simulink library "xbsIndex_r4"  (Simulink 7.1)
(part 6 of 9)

      settings: CopyFcn=xlBlockMoveCallback(gcbh);  DeleteFcn=xlDestroyGui(gcbh);  ModelCloseFcn=xlDestroyGui(gcbh);  PreSaveFcn=xlBlockPreSaveCallback(gcbh);  PostSaveFcn=xlBlockPostSaveCallback(gcbh);  DestroyFcn=xlDestroyGui(gcbh);  OpenFcn=xlOpenGui(gcbh, 'lfsr_gui.xml', @lfsrenablement, -1)  CloseFcn=xlDestroyGui(gcbh);  MoveFcn=xlBlockMoveCallback(gcbh);
      mask Help: eval('');xlDoc('-book','sysgen','-topic','LFSR');
      mask StyleString: edit,popup(Fibonacci|Galois),edit,popup(XOR|XNOR),edit,edit,edit,edit,checkbox,edit,checkbox,edit,checkbox,edit,checkbox,edit,checkbox,edit,popup(Signed  (2's comp)|Unsigned),edit,edit,checkbox,edit,checkbox,edit,edit,checkbox,edit,edit,edit,edit,edit,edit,edit,edit,edit
      mask Display:
      | fprintf('','COMMENT: begin icon graphics');
      | patch([0 60 60 0 0 ],[0 0 60 60 0 ],[0.77 0.82 0.91 ]);
      | plot([0 60 60 0 0 ],[0 0 60 60 0 ]);
      | patch([12.2 23.76 31.76 39.76 47.76 31.76 20.2 12.2 ],[38.88 38.88 46.88 38.88 46.88 46.88 46.88 38.88 ],[1 1 1 ]);
      | patch([20.2 31.76 23.76 12.2 20.2 ],[30.88 30.88 38.88 38.88 30.88 ],[0.931 0.946 0.973 ]);
      | patch([12.2 23.76 31.76 20.2 12.2 ],[22.88 22.88 30.88 30.88 22.88 ],[1 1 1 ]);
      | patch([20.2 47.76 39.76 31.76 23.76 12.2 20.2 ],[14.88 14.88 22.88 14.88 22.88 22.88 14.88 ],[0.931 0.946 0.973 ]);
      | fprintf('','COMMENT: end icon graphics');
      | fprintf('','COMMENT: begin icon text');
      | color('black');port_label('output',1,'dout');
      | fprintf('','COMMENT: end icon text');
  Logical : S-Function  LoadFcn=xlBlockLoadCallback(gcbh);  FunctionName=sysgen  Parameters=ptable_  EnableBusSupport=off  mask(Xilinx Logical Block Block){logical_function_sgadvanced=, logical_function=AND, inputs=2, en_sgadvanced=, en=off, latency=0, precision_sgadvanced=, precision=Full, arith_type_sgadvanced=, arith_type=Unsigned, n_bits=16, bin_pt=0, align_bp_sgadvanced=, align_bp=on, dbl_ovrd_sgadvanced=, dbl_ovrd=off, xl_use_area_sgadvanced=, xl_use_area=off, xl_area=[0,0,0,0,0,0,0], overflow=, quantization=, has_advanced_control=0, sggui_pos=-1,-1,-1,-1, block_type=logical, block_version=, sg_icon_stat=55,60,2,1,white,blue,0,83a4b621,right,,[ ],[ ], sg_mask_display=|, sg_list_contents=, sg_blockgui_xml=}
      mask sg_mask_display=|
      | fprintf('','COMMENT: begin icon graphics');
      | patch([0 55 55 0 0 ],[0 0 60 60 0 ],[0.77 0.82 0.91 ]);
      | plot([0 55 55 0 0 ],[0 0 60 60 0 ]);
      | patch([11.425 21.54 28.54 35.54 42.54 28.54 18.425 11.425 ],[37.77 37.77 44.77 37.77 44.77 44.77 44.77 37.77 ],[1 1 1 ]);
      | patch([18.425 28.54 21.54 11.425 18.425 ],[30.77 30.77 37.77 37.77 30.77 ],[0.931 0.946 0.973 ]);
      | patch([11.425 21.54 28.54 18.425 11.425 ],[23.77 23.77 30.77 30.77 23.77 ],[1 1 1 ]);
      | patch([18.425 42.54 35.54 28.54 21.54 11.425 18.425 ],[16.77 16.77 23.77 16.77 23.77 23.77 16.77 ],[0.931 0.946 0.973 ]);
      | fprintf('','COMMENT: end icon graphics');
      | fprintf('','COMMENT: begin icon text');
      |
      |
      |
      | color('black');disp('and');
      | fprintf('','COMMENT: end icon text');
      mask prompts: logical_function_sgadvanced ""; logical_function "Logical function"; inputs "Number of inputs"; en_sgadvanced ""; en "Provide enable port"; precision_sgadvanced ""; arith_type_sgadvanced ""; arith_type "Output Type"; n_bits "Number of bits"; bin_pt "Binary point"; align_bp_sgadvanced ""; align_bp "Align binary point"; dbl_ovrd_sgadvanced ""; dbl_ovrd "Override with doubles"; xl_use_area_sgadvanced ""; xl_use_area "Define FPGA area for resource estimation"; xl_area "FPGA area [slices, FFs, BRAMs, LUTs, IOBs, emb. mults, TBUFs]"; overflow ""; quantization ""; has_advanced_control ""; sggui_pos ""; block_type ""; block_version ""; sg_icon_stat ""; sg_mask_display ""; sg_list_contents ""; sg_blockgui_xml ""
      mask help: Xilinx Logical Block
      mask init:
      | try
      |   tmp_gcb = gcb;
      |   tmp_gcbh = gcbh;
      |   if (strcmp('SysGenIndex',get_param(bdroot(tmp_gcbh),'tag')) && ~isempty(regexp(bdroot(tmp_gcb), '^xbs', 'once')))
      |     return;
      |   end;
      |   xlMungeMaskParams;
      |   block_config = 'sysgen_blockset:Logical_config';
      | 
      |   block_type='logical';
      | 
      |   serialized_declarations = '{''arith_type''=>''Int'',''bin_pt''=>''Int'',''en''=>''Int'',''inputs''=>''Int'',''latency''=>''Int'',''logical_function''=>''Int'',''n_bits''=>''Int'',''precision''=>''Int'',''sim_engine''=>''Int'',''sysgen_root''=>''String'',''block_type''=>''String''}';
      |   xllogical_init();
      |   ptable_ = xlblockprep(get_param(tmp_gcb, 'MaskWSVariables'));
      |   try
      |     xlBlockMoveCallback(tmp_gcbh);
      |   catch 
      |      clear global xl_updateicon_recursion_guard;
      |   end;
      | catch
      |   global dbgsysgen;
      |   if(~isempty(dbgsysgen) && dbgsysgen)
      |     e = regexprep(lasterr, '\n', '\nError: ');
      |     disp(['Error: While running MaskInit code on block ' tmp_gcb ': ' e]);
      |     error(e);
      |   end
      | end
      settings: CopyFcn=xlBlockMoveCallback(gcbh);  DeleteFcn=xlDestroyGui(gcbh);  ModelCloseFcn=xlDestroyGui(gcbh);  PreSaveFcn=xlBlockPreSaveCallback(gcbh);  PostSaveFcn=xlBlockPostSaveCallback(gcbh);  DestroyFcn=xlDestroyGui(gcbh);  OpenFcn=xlOpenGui(gcbh, 'logical_gui.xml', @logicalenablement, -1)  CloseFcn=xlDestroyGui(gcbh);  MoveFcn=xlBlockMoveCallback(gcbh);
      mask Help: eval('');xlDoc('-book','sysgen','-topic','Logical');
      mask StyleString: edit,popup(AND|NAND|OR|NOR|XOR|XNOR),edit,edit,checkbox,edit,edit,popup(Full|User Defined),edit,popup(Signed  (2's comp)|Unsigned),edit,edit,edit,checkbox,edit,checkbox,edit,checkbox,edit,edit,edit,edit,edit,edit,edit,edit,edit,edit,edit
      mask Display:
      | fprintf('','COMMENT: begin icon graphics');
      | patch([0 55 55 0 0 ],[0 0 60 60 0 ],[0.77 0.82 0.91 ]);
      | plot([0 55 55 0 0 ],[0 0 60 60 0 ]);
      | patch([11.425 21.54 28.54 35.54 42.54 28.54 18.425 11.425 ],[37.77 37.77 44.77 37.77 44.77 44.77 44.77 37.77 ],[1 1 1 ]);
      | patch([18.425 28.54 21.54 11.425 18.425 ],[30.77 30.77 37.77 37.77 30.77 ],[0.931 0.946 0.973 ]);
      | patch([11.425 21.54 28.54 18.425 11.425 ],[23.77 23.77 30.77 30.77 23.77 ],[1 1 1 ]);
      | patch([18.425 42.54 35.54 28.54 21.54 11.425 18.425 ],[16.77 16.77 23.77 16.77 23.77 23.77 16.77 ],[0.931 0.946 0.973 ]);
      | fprintf('','COMMENT: end icon graphics');
      | fprintf('','COMMENT: begin icon text');
      | 
      | 
      | 
      | color('black');disp('and');
      | fprintf('','COMMENT: end icon text');
  MCode : S-Function  LoadFcn=xlBlockLoadCallback(gcbh);  FunctionName=sysgen  Parameters=ptable_  EnableBusSupport=off  mask(Xilinx MCode Block Block){infoedit=Pass input values to a MATLAB function for evaluation in Xilinx fixed-point type. The input ports of the block are input arguments of the function. The output ports of the block are output arguments of the function., mfname=xlmax, explicit_period_sgadvanced=, explicit_period=off, period=1, inputsTable=, outputsTable=, dbl_ovrd_sgadvanced=, dbl_ovrd=off, enable_stdout_sgadvanced=, enable_stdout=off, enable_debug_sgadvanced=, enable_debug=off, xl_use_area_sgadvanced=, xl_use_area=off, xl_area=[0,0,0,0,0,0,0], mfilecontent=, suppress_output=on, defparams={}, hide_port_list={}, has_advanced_control=0, sggui_pos=-1,-1,-1,-1, block_type=mcode, block_version=, sg_icon_stat=65,62,2,1,white,blue,0,0442c75a,right,,[ ],[ ], sg_mask_display=|, sg_list_contents=, sg_blockgui_xml=}
      mask sg_mask_display=|
      | fprintf('','COMMENT: begin icon graphics');
      | patch([0 65 65 0 0 ],[0 0 62 62 0 ],[0.77 0.82 0.91 ]);
      | plot([0 65 65 0 0 ],[0 0 62 62 0 ]);
      | patch([14.2 25.76 33.76 41.76 49.76 33.76 22.2 14.2 ],[39.88 39.88 47.88 39.88 47.88 47.88 47.88 39.88 ],[1 1 1 ]);
      | patch([22.2 33.76 25.76 14.2 22.2 ],[31.88 31.88 39.88 39.88 31.88 ],[0.931 0.946 0.973 ]);
      | patch([14.2 25.76 33.76 22.2 14.2 ],[23.88 23.88 31.88 31.88 23.88 ],[1 1 1 ]);
      | patch([22.2 49.76 41.76 33.76 25.76 14.2 22.2 ],[15.88 15.88 23.88 15.88 23.88 23.88 15.88 ],[0.931 0.946 0.973 ]);
      | fprintf('','COMMENT: end icon graphics');
      | fprintf('','COMMENT: begin icon text');
      | color('black');port_label('input',1,'x');
      | color('black');port_label('input',2,'y');
      | color('black');port_label('output',1,'z');
      | color('black');disp('\bf{xlmax}','texmode','on');
      | fprintf('','COMMENT: end icon text');
      mask prompts: infoedit ""; mfname "MATLAB function"; explicit_period_sgadvanced ""; explicit_period "Specify explicit sample period"; period ""; inputsTable ""; outputsTable ""; dbl_ovrd_sgadvanced ""; dbl_ovrd "Override with doubles"; enable_stdout_sgadvanced ""; enable_stdout "Enable printing with disp"; enable_debug_sgadvanced ""; enable_debug "Enable MATLAB debugging (slows simulation)"; xl_use_area_sgadvanced ""; xl_use_area "Define FPGA area for resource estimation"; xl_area "FPGA area [slices, FFs, BRAMs, LUTs, IOBs, emb. mults, TBUFs]"; mfilecontent ""; suppress_output ""; defparams ""; hide_port_list ""; has_advanced_control ""; sggui_pos ""; block_type ""; block_version ""; sg_icon_stat ""; sg_mask_display ""; sg_list_contents ""; sg_blockgui_xml ""
      mask help: Pass input values to a MATLAB function for evaluation in Xilinx fixed-point type. The input ports of the block are input arguments of the function. The output ports of the block are output arguments of the function.
      mask init:
      | try
      |   tmp_gcb = gcb;
      |   tmp_gcbh = gcbh;
      |   if (strcmp('SysGenIndex',get_param(bdroot(tmp_gcbh),'tag')) && ~isempty(regexp(bdroot(tmp_gcb), '^xbs', 'once')))
      |     return;
      |   end;
      |   xlMungeMaskParams;
      |   block_config = 'sysgen_blockset:mcode_block_config';
      | 
      |   block_type='mcode';
      | 
      |   serialized_declarations = '{''block_fullname''=>''String'',''bool_vec_lens''=>''IntVector'',''bool_vec_names''=>''StringVector'',''bool_vec_values''=>''IntVector'',''dbl_vec_lens''=>''IntVector'',''dbl_vec_names''=>''StringVector'',''dbl_vec_values''=>''DoubleVector'',''defparams''=>''Struct'',''drawport''=>''String'',''enable_debug''=>''Int'',''enable_stdout''=>''Int'',''error_msgs''=>''StringVector'',''explicitClk''=>''Int'',''explicit_period''=>''Int'',''hide_port_list''=>''StringVector'',''icontext''=>''String'',''mfile_dir''=>''String'',''mfilecontent''=>''String'',''mfilename''=>''String'',''mfname''=>''String'',''param_names_bool''=>''StringVector'',''param_names_double''=>''StringVector'',''param_values_bool''=>''IntVector'',''param_values_double''=>''DoubleVector'',''period''=>''Double'',''sgpfilename''=>''String'',''sysgen_root''=>''String'',''block_type''=>''String''}';
      |   xlmcode_init();
      |   ptable_ = xlblockprep(get_param(tmp_gcb, 'MaskWSVariables'));
      |   try
      |     xlBlockMoveCallback(tmp_gcbh);
      |   catch 
      |      clear global xl_updateicon_recursion_guard;
      |   end;
      | catch
      |   global dbgsysgen;
      |   if(~isempty(dbgsysgen) && dbgsysgen)
      |     e = regexprep(lasterr, '\n', '\nError: ');
      |     disp(['Error: While running MaskInit code on block ' tmp_gcb ': ' e]);
      |     error(e);
      |   end
      | end
      settings: CopyFcn=xlBlockMoveCallback(gcbh);  DeleteFcn=xlDestroyGui(gcbh);  ModelCloseFcn=xlDestroyGui(gcbh);  PreSaveFcn=xlBlockPreSaveCallback(gcbh);  PostSaveFcn=xlBlockPostSaveCallback(gcbh);  DestroyFcn=xlDestroyGui(gcbh);  OpenFcn=xlOpenGui(gcbh, 'mcode_gui.xml', @mcodeenablement, @mcodeaction)  CloseFcn=xlDestroyGui(gcbh);  MoveFcn=xlBlockMoveCallback(gcbh);
      mask Help: eval('');xlDoc('-book','sysgen','-topic','MCode');
      mask Display:
      | fprintf('','COMMENT: begin icon graphics');
      | patch([0 65 65 0 0 ],[0 0 62 62 0 ],[0.77 0.82 0.91 ]);
      | plot([0 65 65 0 0 ],[0 0 62 62 0 ]);
      | patch([14.2 25.76 33.76 41.76 49.76 33.76 22.2 14.2 ],[39.88 39.88 47.88 39.88 47.88 47.88 47.88 39.88 ],[1 1 1 ]);
      | patch([22.2 33.76 25.76 14.2 22.2 ],[31.88 31.88 39.88 39.88 31.88 ],[0.931 0.946 0.973 ]);
      | patch([14.2 25.76 33.76 22.2 14.2 ],[23.88 23.88 31.88 31.88 23.88 ],[1 1 1 ]);
      | patch([22.2 49.76 41.76 33.76 25.76 14.2 22.2 ],[15.88 15.88 23.88 15.88 23.88 23.88 15.88 ],[0.931 0.946 0.973 ]);
      | fprintf('','COMMENT: end icon graphics');
      | fprintf('','COMMENT: begin icon text');
      | color('black');port_label('input',1,'x');
      | color('black');port_label('input',2,'y');
      | color('black');port_label('output',1,'z');
      | color('black');disp('\bf{xlmax}','texmode','on');
      | fprintf('','COMMENT: end icon text');
  ModelSim : S-Function  LoadFcn=xlBlockLoadCallback(gcbh);  FunctionName=sysgen  Parameters=ptable_  EnableBusSupport=off  mask(ModelSim HDL Co-Simulation Interface Block){infoedit=Allow other blocks to schedule HDL co-simulation tasks.<br><br>Note that selecting "Skip compilation" when inappropriate can cause simulation errors and failures. Please refer to the block help for details., dir=./modelsim, waveform_sgadvanced=, waveform=on, leave_open_sgadvanced=, leave_open=on, skip_compile_sgadvanced=, skip_compile=off, use_unisim_sgadvanced=, use_unisim=off, use_ver_xilinxcorelib_sgadvanced=, use_ver_xilinxcorelib=off, custom_scripts_sgadvanced=, custom_scripts=off, pre_comp_script=, vsim_script=, post_vsim_script=, startup_timeout=40, has_advanced_control=0, sggui_pos=-1,-1,-1,-1, block_type=hdlcosim, block_version=, sg_icon_stat=65,56,0,0,blue,white,0,efd5b770,right,,[ ],[ ], sg_mask_display=|, sg_list_contents=, sg_blockgui_xml=}
      mask sg_mask_display=|
      | fprintf('','COMMENT: begin icon graphics');
      | patch([0 65 65 0 0 ],[0 0 56 56 0 ],[1 1 1 ]);
      | plot([0 65 65 0 0 ],[0 0 56 56 0 ]);
      | patch([14.2 25.76 33.76 41.76 49.76 33.76 22.2 14.2 ],[36.88 36.88 44.88 36.88 44.88 44.88 44.88 36.88 ],[0.839 0.874 0.937 ]);
      | patch([22.2 33.76 25.76 14.2 22.2 ],[28.88 28.88 36.88 36.88 28.88 ],[0.77 0.82 0.91 ]);
      | patch([14.2 25.76 33.76 22.2 14.2 ],[20.88 20.88 28.88 28.88 20.88 ],[0.839 0.874 0.937 ]);
      | patch([22.2 49.76 41.76 33.76 25.76 14.2 22.2 ],[12.88 12.88 20.88 12.88 20.88 20.88 12.88 ],[0.77 0.82 0.91 ]);
      | fprintf('','COMMENT: end icon graphics');
      | fprintf('','COMMENT: begin icon text');
      |
      | fprintf('','COMMENT: end icon text');fprintf('ModelSim');
      mask prompts: infoedit ""; dir "Run co-simulation in directory:"; waveform_sgadvanced ""; waveform "Open waveform viewer"; leave_open_sgadvanced ""; leave_open "Leave ModelSim open at end of simulation"; skip_compile_sgadvanced ""; skip_compile "Skip compilation (use previous results)"; use_unisim_sgadvanced ""; use_unisim "Include Verilog unisim library"; use_ver_xilinxcorelib_sgadvanced ""; use_ver_xilinxcorelib "Include Verilog XILINXCORELIB library"; custom_scripts_sgadvanced ""; custom_scripts "Add custom scripts"; pre_comp_script "Script to run before starting compilation:"; vsim_script "Script to run in place of  "vsim":"; post_vsim_script "Script to run after "vsim":"; startup_timeout ""; has_advanced_control ""; sggui_pos ""; block_type ""; block_version ""; sg_icon_stat ""; sg_mask_display ""; sg_list_contents ""; sg_blockgui_xml ""
      mask help:
      | Allow other blocks to schedule HDL co-simulation tasks.
      |
      | Note that selecting "Skip compilation" when inappropriate can cause simulation errors and failures. Please refer to the block help for details.
      mask init:
      | try
      |   tmp_gcb = gcb;
      |   tmp_gcbh = gcbh;
      |   if (strcmp('SysGenIndex',get_param(bdroot(tmp_gcbh),'tag')) && ~isempty(regexp(bdroot(tmp_gcb), '^xbs', 'once')))
      |     return;
      |   end;
      |   xlMungeMaskParams;
      |   block_config = 'Sysgen:hdlcosim_block_config';
      | 
      |   block_type='hdlcosim';
      | 
      |   serialized_declarations = '{''binDir''=>''String'',''custom_scripts''=>''Int'',''dir''=>''String'',''engineDll''=>''String'',''leave_open''=>''Int'',''mdlPath''=>''String'',''period''=>''Double'',''post_vsim_script''=>''String'',''pre_comp_script''=>''String'',''screenSize''=>''DoubleVector'',''sim_status''=>''String'',''skip_compile''=>''Int'',''startup_timeout''=>''Int'',''use_unisim''=>''Int'',''use_ver_xilinxcorelib''=>''Int'',''vsim_script''=>''String'',''waveform''=>''Int'',''block_type''=>''String''}';
      |   xlhdlcosim_init();
      |   ptable_ = xlblockprep(get_param(tmp_gcb, 'MaskWSVariables'));
      |   try
      |     xlBlockMoveCallback(tmp_gcbh);
      |   catch 
      |      clear global xl_updateicon_recursion_guard;
      |   end;
      | catch
      |   global dbgsysgen;
      |   if(~isempty(dbgsysgen) && dbgsysgen)
      |     e = regexprep(lasterr, '\n', '\nError: ');
      |     disp(['Error: While running MaskInit code on block ' tmp_gcb ': ' e]);
      |     error(e);
      |   end
      | end
      settings: CopyFcn=xlBlockMoveCallback(gcbh);  DeleteFcn=xlDestroyGui(gcbh);  ModelCloseFcn=xlDestroyGui(gcbh);  PreSaveFcn=xlBlockPreSaveCallback(gcbh);  PostSaveFcn=xlBlockPostSaveCallback(gcbh);  DestroyFcn=xlDestroyGui(gcbh);  OpenFcn=xlOpenGui(gcbh, 'hdlcosim_gui.xml', @hdlcosimenablement, -1)  CloseFcn=xlDestroyGui(gcbh);  MoveFcn=xlBlockMoveCallback(gcbh);
      mask Help: eval('');xlDoc('-book','sysgen','-topic','ModelSim');
      mask Display:
      | fprintf('','COMMENT: begin icon graphics');
      | patch([0 65 65 0 0 ],[0 0 56 56 0 ],[1 1 1 ]);
      | plot([0 65 65 0 0 ],[0 0 56 56 0 ]);
      | patch([14.2 25.76 33.76 41.76 49.76 33.76 22.2 14.2 ],[36.88 36.88 44.88 36.88 44.88 44.88 44.88 36.88 ],[0.839 0.874 0.937 ]);
      | patch([22.2 33.76 25.76 14.2 22.2 ],[28.88 28.88 36.88 36.88 28.88 ],[0.77 0.82 0.91 ]);
      | patch([14.2 25.76 33.76 22.2 14.2 ],[20.88 20.88 28.88 28.88 20.88 ],[0.839 0.874 0.937 ]);
      | patch([22.2 49.76 41.76 33.76 25.76 14.2 22.2 ],[12.88 12.88 20.88 12.88 20.88 20.88 12.88 ],[0.77 0.82 0.91 ]);
      | fprintf('','COMMENT: end icon graphics');
      | fprintf('','COMMENT: begin icon text');
      | 
      | fprintf('','COMMENT: end icon text');fprintf('ModelSim');
  Mult : S-Function  LoadFcn=xlBlockLoadCallback(gcbh);  FunctionName=sysgen  Parameters=ptable_  EnableBusSupport=off  mask(Xilinx Multiplier Block){infoedit=Hardware notes: To check for the optimum internal pipeline stages of the dedicated multiplier you must select 'Test for optimum pipelining'.<br><br>Optimization Goal: For implementation into device fabric (LUTs), the Speed or Area optimization will take effect only if it's supported by IP for the particular device family. Otherwise, the results will be identical regardless of the selection., precision_sgadvanced=, precision=Full, arith_type_sgadvanced=, arith_type=Signed  (2's comp), n_bits=16, bin_pt=14, quantization_sgadvanced=, quantization=Truncate, overflow_sgadvanced=, overflow=Wrap, en_sgadvanced=, en=off, latency=3, dbl_ovrd_sgadvanced=, dbl_ovrd=off, use_behavioral_HDL_sgadvanced=, use_behavioral_HDL=off, opt_sgadvanced=, opt=Speed, use_embedded_sgadvanced=, use_embedded=on, optimum_pipeline_sgadvanced=, optimum_pipeline=off, xl_use_area_sgadvanced=, xl_use_area=off, xl_area=[0,0,0,0,0,0,0], pipeline=on, use_rpm=on, placement_style=Triangular, has_advanced_control=0, sggui_pos=-1,-1,-1,-1, block_type=mult, block_version=, sg_icon_stat=55,55,2,1,white,blue,0,7028354c,right,,[ ],[ ], sg_mask_display=|, sg_list_contents=, sg_blockgui_xml=}
      mask sg_mask_display=|
      | fprintf('','COMMENT: begin icon graphics');
      | patch([0 55 55 0 0 ],[0 0 55 55 0 ],[0.77 0.82 0.91 ]);
      | plot([0 55 55 0 0 ],[0 0 55 55 0 ]);
      | patch([11.425 21.54 28.54 35.54 42.54 28.54 18.425 11.425 ],[34.77 34.77 41.77 34.77 41.77 41.77 41.77 34.77 ],[1 1 1 ]);
      | patch([18.425 28.54 21.54 11.425 18.425 ],[27.77 27.77 34.77 34.77 27.77 ],[0.931 0.946 0.973 ]);
      | patch([11.425 21.54 28.54 18.425 11.425 ],[20.77 20.77 27.77 27.77 20.77 ],[1 1 1 ]);
      | patch([18.425 42.54 35.54 28.54 21.54 11.425 18.425 ],[13.77 13.77 20.77 13.77 20.77 20.77 13.77 ],[0.931 0.946 0.973 ]);
      | fprintf('','COMMENT: end icon graphics');
      | fprintf('','COMMENT: begin icon text');
      | color('black');port_label('input',1,'a');
      | color('black');port_label('input',2,'b');
      | color('black');port_label('output',1,'\bfa \times b','texmode','on');
      | color('black');disp('z^{-3}\newline ','texmode','on');
      | color('black');disp(' \n ');
      | fprintf('','COMMENT: end icon text');
      mask prompts: infoedit ""; precision_sgadvanced ""; arith_type_sgadvanced ""; arith_type "Arithmetic type"; n_bits "Number of bits"; bin_pt "Binary point"; quantization_sgadvanced ""; overflow_sgadvanced ""; en_sgadvanced ""; en "Provide enable port"; dbl_ovrd_sgadvanced ""; dbl_ovrd "Override with doubles"; use_behavioral_HDL_sgadvanced ""; use_behavioral_HDL "Use behavioral HDL (otherwise use core)"; opt_sgadvanced ""; opt "Optimize for"; use_embedded_sgadvanced ""; use_embedded "Use embedded multipliers"; optimum_pipeline_sgadvanced ""; optimum_pipeline "Test for optimum pipelining"; xl_use_area_sgadvanced ""; xl_use_area "Define FPGA area for resource estimation"; xl_area "FPGA area [slices, FFs, BRAMs, LUTs, IOBs, emb. mults, TBUFs]"; pipeline ""; use_rpm ""; placement_style ""; has_advanced_control ""; sggui_pos ""; block_type ""; block_version ""; sg_icon_stat ""; sg_mask_display ""; sg_list_contents ""; sg_blockgui_xml ""
      mask help:
      | Hardware notes: To check for the optimum internal pipeline stages of the dedicated multiplier you must select 'Test for optimum pipelining'.
      |
      | Optimization Goal: For implementation into device fabric (LUTs), the Speed or Area optimization will take effect only if it's supported by IP for the particular device family. Otherwise, the results will be identical regardless of the selection.
      mask init:
      | try
      |   tmp_gcb = gcb;
      |   tmp_gcbh = gcbh;
      |   if (strcmp('SysGenIndex',get_param(bdroot(tmp_gcbh),'tag')) && ~isempty(regexp(bdroot(tmp_gcb), '^xbs', 'once')))
      |     return;
      |   end;
      |   xlMungeMaskParams;
      |   block_config = 'sysgen_blockset:Mult_config';
      | 
      |   block_type='mult';
      | 
      |   serialized_declarations = '{''arith_type''=>''Int'',''bin_pt''=>''Int'',''en''=>''Int'',''latency''=>''Int'',''n_bits''=>''Int'',''opt''=>''Int'',''optimum_pipeline''=>''Int'',''overflow''=>''Int'',''precision''=>''Int'',''quantization''=>''Int'',''use_behavioral_HDL''=>''Int'',''use_embedded''=>''Int'',''block_type''=>''String''}';
      |   ptable_ = xlblockprep(get_param(tmp_gcb, 'MaskWSVariables'));
      |   try
      |     xlBlockMoveCallback(tmp_gcbh);
      |   catch 
      |      clear global xl_updateicon_recursion_guard;
      |   end;
      | catch
      |   global dbgsysgen;
      |   if(~isempty(dbgsysgen) && dbgsysgen)
      |     e = regexprep(lasterr, '\n', '\nError: ');
      |     disp(['Error: While running MaskInit code on block ' tmp_gcb ': ' e]);
      |     error(e);
      |   end
      | end
      settings: CopyFcn=xlBlockMoveCallback(gcbh);  DeleteFcn=xlDestroyGui(gcbh);  ModelCloseFcn=xlDestroyGui(gcbh);  PreSaveFcn=xlBlockPreSaveCallback(gcbh);  PostSaveFcn=xlBlockPostSaveCallback(gcbh);  DestroyFcn=xlDestroyGui(gcbh);  OpenFcn=xlOpenGui(gcbh, 'mult_gui.xml', @multenablement, -1)  CloseFcn=xlDestroyGui(gcbh);  MoveFcn=xlBlockMoveCallback(gcbh);
      mask Help: eval('');xlDoc('-book','sysgen','-topic','Mult');
      mask StyleString: edit,edit,popup(Full|User Defined),edit,popup(Signed  (2's comp)|Unsigned),edit,edit,edit,popup(Truncate|Round  (unbiased: +/- Inf)),edit,popup(Wrap|Saturate|Flag as error),edit,checkbox,edit,edit,checkbox,edit,checkbox,edit,popup(Speed|Area),edit,checkbox,edit,checkbox,edit,checkbox,edit,edit,edit,edit,edit,edit,edit,edit,edit,edit,edit,edit
      mask Display:
      | fprintf('','COMMENT: begin icon graphics');
      | patch([0 55 55 0 0 ],[0 0 55 55 0 ],[0.77 0.82 0.91 ]);
      | plot([0 55 55 0 0 ],[0 0 55 55 0 ]);
      | patch([11.425 21.54 28.54 35.54 42.54 28.54 18.425 11.425 ],[34.77 34.77 41.77 34.77 41.77 41.77 41.77 34.77 ],[1 1 1 ]);
      | patch([18.425 28.54 21.54 11.425 18.425 ],[27.77 27.77 34.77 34.77 27.77 ],[0.931 0.946 0.973 ]);
      | patch([11.425 21.54 28.54 18.425 11.425 ],[20.77 20.77 27.77 27.77 20.77 ],[1 1 1 ]);
      | patch([18.425 42.54 35.54 28.54 21.54 11.425 18.425 ],[13.77 13.77 20.77 13.77 20.77 20.77 13.77 ],[0.931 0.946 0.973 ]);
      | fprintf('','COMMENT: end icon graphics');
      | fprintf('','COMMENT: begin icon text');
      | color('black');port_label('input',1,'a');
      | color('black');port_label('input',2,'b');
      | color('black');port_label('output',1,'\bfa \times b','texmode','on');
      | color('black');disp('z^{-3}\newline ','texmode','on');
      | color('black');disp(' \n ');
      | fprintf('','COMMENT: end icon text');
  Multiple Subsystem Generator : S-Function  Tag=xlStitcher  FunctionName=xlpermissive  Parameters=''  EnableBusSupport=off  mask(Xilinx Subsystem Generator Block){infoedit=Multiple Subsystem\nGenerator, ShowPortLabels=, has_advanced_control=0, sggui_pos=-1,-1,-1,-1, block_type=multiple_subsystem_generator, block_version=, sg_icon_stat=65,65,-1,-1,blue,white,0,07734,right,,[ ],[ ], sg_mask_display=|, sg_list_contents=, sg_blockgui_xml=}
      mask sg_mask_display=|
      | fprintf('','COMMENT: begin icon graphics');
      | patch([0 65 65 0 0 ],[0 0 65 65 0 ],[1 1 1 ]);
      | plot([0 65 65 0 0 ],[0 0 65 65 0 ]);
      | patch([11.975 24.98 33.98 42.98 51.98 33.98 20.975 11.975 ],[41.99 41.99 50.99 41.99 50.99 50.99 50.99 41.99 ],[0.839 0.874 0.937 ]);
      | patch([20.975 33.98 24.98 11.975 20.975 ],[32.99 32.99 41.99 41.99 32.99 ],[0.77 0.82 0.91 ]);
      | patch([11.975 24.98 33.98 20.975 11.975 ],[23.99 23.99 32.99 32.99 23.99 ],[0.839 0.874 0.937 ]);
      | patch([20.975 51.98 42.98 33.98 24.98 11.975 20.975 ],[14.99 14.99 23.99 14.99 23.99 23.99 14.99 ],[0.77 0.82 0.91 ]);
      | fprintf('','COMMENT: end icon graphics');
      | fprintf('','COMMENT: begin icon text');
      | fprintf('','COMMENT: end icon text');
      mask prompts: infoedit ""; ShowPortLabels ""; has_advanced_control ""; sggui_pos ""; block_type ""; block_version ""; sg_icon_stat ""; sg_mask_display ""; sg_list_contents ""; sg_blockgui_xml ""
      mask help: Multiple Subsystem\nGenerator
      mask init:
      | try
      |   tmp_gcb = gcb;
      |   tmp_gcbh = gcbh;
      |   if (strcmp('SysGenIndex',get_param(bdroot(tmp_gcbh),'tag')) && ~isempty(regexp(bdroot(tmp_gcb), '^xbs', 'once')))
      |     return;
      |   end;
      |   xlMungeMaskParams;
      | 
      |   block_type='multiple_subsystem_generator';
      | 
      |   serialized_declarations = '{''block_type''=>''String''}';
      |   ptable_ = xlblockprep(get_param(tmp_gcb, 'MaskWSVariables'));
      |   try
      |     xlBlockMoveCallback(tmp_gcbh);
      |   catch 
      |      clear global xl_updateicon_recursion_guard;
      |   end;
      | catch
      |   global dbgsysgen;
      |   if(~isempty(dbgsysgen) && dbgsysgen)
      |     e = regexprep(lasterr, '\n', '\nError: ');
      |     disp(['Error: While running MaskInit code on block ' tmp_gcb ': ' e]);
      |     error(e);
      |   end
      | end
      settings: CopyFcn=xlBlockMoveCallback(gcbh);  OpenFcn=xldesignStitcher(gcbh);  MoveFcn=xlBlockMoveCallback(gcbh);
      settings: DeleteFcn=|
      | hndls = xlfindsysgenfig(gcb,'stitcher_gui');
      | if (hndls)
      |   close(hndls(1));
      | end
      mask Help: eval('');xlDoc('-book','sysgen','-topic','Multiple_Subsystem_Generator');
      mask Display:
      | fprintf('','COMMENT: begin icon graphics');
      | patch([0 65 65 0 0 ],[0 0 65 65 0 ],[1 1 1 ]);
      | plot([0 65 65 0 0 ],[0 0 65 65 0 ]);
      | patch([11.975 24.98 33.98 42.98 51.98 33.98 20.975 11.975 ],[41.99 41.99 50.99 41.99 50.99 50.99 50.99 41.99 ],[0.839 0.874 0.937 ]);
      | patch([20.975 33.98 24.98 11.975 20.975 ],[32.99 32.99 41.99 41.99 32.99 ],[0.77 0.82 0.91 ]);
      | patch([11.975 24.98 33.98 20.975 11.975 ],[23.99 23.99 32.99 32.99 23.99 ],[0.839 0.874 0.937 ]);
      | patch([20.975 51.98 42.98 33.98 24.98 11.975 20.975 ],[14.99 14.99 23.99 14.99 23.99 23.99 14.99 ],[0.77 0.82 0.91 ]);
      | fprintf('','COMMENT: end icon graphics');
      | fprintf('','COMMENT: begin icon text');
      | fprintf('','COMMENT: end icon text');
  Mux : S-Function  LoadFcn=xlBlockLoadCallback(gcbh);  FunctionName=sysgen  Parameters=ptable_  EnableBusSupport=off  mask(Xilinx Bus Multiplexer Block){inputs_sgadvanced=, inputs=2, en_sgadvanced=, en=off, latency=0, precision_sgadvanced=, precision=Full, arith_type_sgadvanced=, arith_type=Unsigned, n_bits=16, bin_pt=14, quantization_sgadvanced=, quantization=Truncate, overflow_sgadvanced=, overflow=Wrap, dbl_ovrd_sgadvanced=, dbl_ovrd=off, xl_use_area_sgadvanced=, xl_use_area=off, xl_area=[0,0,0,0,0,0,0], infoedit=, has_advanced_control=0, sggui_pos=-1,-1,-1,-1, block_type=mux, block_version=, sg_icon_stat=45,104,3,1,white,blue,3,eb98d690,right,,[ ],[ ], sg_mask_display=|, sg_list_contents=, sg_blockgui_xml=}
      mask sg_mask_display=|
      | fprintf('','COMMENT: begin icon graphics');
      | patch([0 45 45 0 0 ],[0 14.8571 89.1429 104 0 ],[0.77 0.82 0.91 ]);
      | plot([0 45 45 0 0 ],[0 14.8571 89.1429 104 0 ]);
      | patch([8.65 17.32 23.32 29.32 35.32 23.32 14.65 8.65 ],[58.66 58.66 64.66 58.66 64.66 64.66 64.66 58.66 ],[1 1 1 ]);
      | patch([14.65 23.32 17.32 8.65 14.65 ],[52.66 52.66 58.66 58.66 52.66 ],[0.931 0.946 0.973 ]);
      | patch([8.65 17.32 23.32 14.65 8.65 ],[46.66 46.66 52.66 52.66 46.66 ],[1 1 1 ]);
      | patch([14.65 35.32 29.32 23.32 17.32 8.65 14.65 ],[40.66 40.66 46.66 40.66 46.66 46.66 40.66 ],[0.931 0.946 0.973 ]);
      | fprintf('','COMMENT: end icon graphics');
      | fprintf('','COMMENT: begin icon text');
      | color('black');port_label('input',1,'sel');
      | color('black');port_label('input',2,'d0');
      | color('black');port_label('input',3,'d1');
      |
      | color('black');disp('\bf{}','texmode','on');
      | fprintf('','COMMENT: end icon text');
      mask prompts: inputs_sgadvanced ""; inputs "Number of inputs"; en_sgadvanced ""; en "Provide enable port"; precision_sgadvanced ""; arith_type_sgadvanced ""; arith_type "Arithmetic type"; n_bits "Number of bits"; bin_pt "Binary point"; quantization_sgadvanced ""; overflow_sgadvanced ""; dbl_ovrd_sgadvanced ""; dbl_ovrd "Override with doubles"; xl_use_area_sgadvanced ""; xl_use_area "Define FPGA area for resource estimation"; xl_area "FPGA area [slices, FFs, BRAMs, LUTs, IOBs, emb. mults, TBUFs]"; infoedit ""; has_advanced_control ""; sggui_pos ""; block_type ""; block_version ""; sg_icon_stat ""; sg_mask_display ""; sg_list_contents ""; sg_blockgui_xml ""
      mask help: Xilinx Bus Multiplexer
      mask init:
      | try
      |   tmp_gcb = gcb;
      |   tmp_gcbh = gcbh;
      |   if (strcmp('SysGenIndex',get_param(bdroot(tmp_gcbh),'tag')) && ~isempty(regexp(bdroot(tmp_gcb), '^xbs', 'once')))
      |     return;
      |   end;
      |   xlMungeMaskParams;
      |   block_config = 'sysgen_blockset:Mux_config';
      | 
      |   block_type='mux';
      | 
      |   serialized_declarations = '{''arith_type''=>''Int'',''bin_pt''=>''Int'',''dbl_ovrd''=>''Int'',''en''=>''Int'',''inputs''=>''Int'',''latency''=>''Int'',''n_bits''=>''Int'',''overflow''=>''Int'',''period''=>''Double'',''precision''=>''Int'',''quantization''=>''Int'',''sim_engine''=>''Int'',''sysgen_root''=>''String'',''block_type''=>''String''}';
      |   xlmux_init();
      |   ptable_ = xlblockprep(get_param(tmp_gcb, 'MaskWSVariables'));
      |   try
      |     xlBlockMoveCallback(tmp_gcbh);
      |   catch 
      |      clear global xl_updateicon_recursion_guard;
      |   end;
      | catch
      |   global dbgsysgen;
      |   if(~isempty(dbgsysgen) && dbgsysgen)
      |     e = regexprep(lasterr, '\n', '\nError: ');
      |     disp(['Error: While running MaskInit code on block ' tmp_gcb ': ' e]);
      |     error(e);
      |   end
      | end
      settings: CopyFcn=xlBlockMoveCallback(gcbh);  DeleteFcn=xlDestroyGui(gcbh);  ModelCloseFcn=xlDestroyGui(gcbh);  PreSaveFcn=xlBlockPreSaveCallback(gcbh);  PostSaveFcn=xlBlockPostSaveCallback(gcbh);  DestroyFcn=xlDestroyGui(gcbh);  OpenFcn=xlOpenGui(gcbh, 'mux_gui.xml', @muxenablement, -1)  CloseFcn=xlDestroyGui(gcbh);  MoveFcn=xlBlockMoveCallback(gcbh);
      mask Help: eval('');xlDoc('-book','sysgen','-topic','Mux');
      mask StyleString: edit,popup(2|3|4|5|6|7|8|9|10|11|12|13|14|15|16|17|18|19|20|21|22|23|24|25|26|27|28|29|30|31|32),edit,checkbox,edit,edit,popup(Full|User Defined),edit,popup(Signed  (2's comp)|Unsigned),edit,edit,edit,popup(Truncate|Round  (unbiased: +/- Inf)),edit,popup(Wrap|Saturate|Flag as error),edit,checkbox,edit,checkbox,edit,edit,edit,edit,edit,edit,edit,edit,edit,edit
      mask Display:
      | fprintf('','COMMENT: begin icon graphics');
      | patch([0 45 45 0 0 ],[0 14.8571 89.1429 104 0 ],[0.77 0.82 0.91 ]);
      | plot([0 45 45 0 0 ],[0 14.8571 89.1429 104 0 ]);
      | patch([8.65 17.32 23.32 29.32 35.32 23.32 14.65 8.65 ],[58.66 58.66 64.66 58.66 64.66 64.66 64.66 58.66 ],[1 1 1 ]);
      | patch([14.65 23.32 17.32 8.65 14.65 ],[52.66 52.66 58.66 58.66 52.66 ],[0.931 0.946 0.973 ]);
      | patch([8.65 17.32 23.32 14.65 8.65 ],[46.66 46.66 52.66 52.66 46.66 ],[1 1 1 ]);
      | patch([14.65 35.32 29.32 23.32 17.32 8.65 14.65 ],[40.66 40.66 46.66 40.66 46.66 46.66 40.66 ],[0.931 0.946 0.973 ]);
      | fprintf('','COMMENT: end icon graphics');
      | fprintf('','COMMENT: begin icon text');
      | color('black');port_label('input',1,'sel');
      | color('black');port_label('input',2,'d0');
      | color('black');port_label('input',3,'d1');
      | 
      | color('black');disp('\bf{}','texmode','on');
      | fprintf('','COMMENT: end icon text');
  Negate : S-Function  LoadFcn=xlBlockLoadCallback(gcbh);  FunctionName=sysgen  Parameters=ptable_  EnableBusSupport=off  mask(Xilinx Negate Block Block){precision_sgadvanced=, precision=Full, arith_type_sgadvanced=, arith_type=Unsigned, n_bits=16, bin_pt=14, quantization_sgadvanced=, quantization=Truncate, overflow_sgadvanced=, overflow=Wrap, en_sgadvanced=, en=off, latency=0, dbl_ovrd_sgadvanced=, dbl_ovrd=off, xl_use_area_sgadvanced=, xl_use_area=off, xl_area=[0,0,0,0,0,0,0], has_advanced_control=0, sggui_pos=-1,-1,-1,-1, block_type=negate, block_version=, sg_icon_stat=55,56,1,1,white,blue,0,36bd7045,right,,[ ],[ ], sg_mask_display=|, sg_list_contents=, sg_blockgui_xml=}
      mask sg_mask_display=|
      | fprintf('','COMMENT: begin icon graphics');
      | patch([0 55 55 0 0 ],[0 0 56 56 0 ],[0.77 0.82 0.91 ]);
      | plot([0 55 55 0 0 ],[0 0 56 56 0 ]);
      | patch([11.425 21.54 28.54 35.54 42.54 28.54 18.425 11.425 ],[35.77 35.77 42.77 35.77 42.77 42.77 42.77 35.77 ],[1 1 1 ]);
      | patch([18.425 28.54 21.54 11.425 18.425 ],[28.77 28.77 35.77 35.77 28.77 ],[0.931 0.946 0.973 ]);
      | patch([11.425 21.54 28.54 18.425 11.425 ],[21.77 21.77 28.77 28.77 21.77 ],[1 1 1 ]);
      | patch([18.425 42.54 35.54 28.54 21.54 11.425 18.425 ],[14.77 14.77 21.77 14.77 21.77 21.77 14.77 ],[0.931 0.946 0.973 ]);
      | fprintf('','COMMENT: end icon graphics');
      | fprintf('','COMMENT: begin icon text');
      |
      |
      | color('black');disp('\bf{x(-1)}','texmode','on');
      | fprintf('','COMMENT: end icon text');
      mask prompts: precision_sgadvanced ""; arith_type_sgadvanced ""; arith_type "Arithmetic type"; n_bits "Number of bits"; bin_pt "Binary point"; quantization_sgadvanced ""; overflow_sgadvanced ""; en_sgadvanced ""; en "Provide enable port"; dbl_ovrd_sgadvanced ""; dbl_ovrd "Override with doubles"; xl_use_area_sgadvanced ""; xl_use_area "Define FPGA area for resource estimation"; xl_area "FPGA area [slices, FFs, BRAMs, LUTs, IOBs, emb. mults, TBUFs]"; has_advanced_control ""; sggui_pos ""; block_type ""; block_version ""; sg_icon_stat ""; sg_mask_display ""; sg_list_contents ""; sg_blockgui_xml ""
      mask help: Xilinx Negate Block
      mask init:
      | try
      |   tmp_gcb = gcb;
      |   tmp_gcbh = gcbh;
      |   if (strcmp('SysGenIndex',get_param(bdroot(tmp_gcbh),'tag')) && ~isempty(regexp(bdroot(tmp_gcb), '^xbs', 'once')))
      |     return;
      |   end;
      |   xlMungeMaskParams;
      |   block_config = 'sysgen_blockset:Negate_config';
      | 
      |   block_type='negate';
      | 
      |   serialized_declarations = '{''arith_type''=>''Int'',''bin_pt''=>''Int'',''dbl_ovrd''=>''Int'',''en''=>''Int'',''latency''=>''Int'',''n_bits''=>''Int'',''overflow''=>''Int'',''precision''=>''Int'',''quantization''=>''Int'',''rst''=>''Int'',''block_type''=>''String''}';
      |   ptable_ = xlblockprep(get_param(tmp_gcb, 'MaskWSVariables'));
      |   try
      |     xlBlockMoveCallback(tmp_gcbh);
      |   catch 
      |      clear global xl_updateicon_recursion_guard;
      |   end;
      | catch
      |   global dbgsysgen;
      |   if(~isempty(dbgsysgen) && dbgsysgen)
      |     e = regexprep(lasterr, '\n', '\nError: ');
      |     disp(['Error: While running MaskInit code on block ' tmp_gcb ': ' e]);
      |     error(e);
      |   end
      | end
      settings: CopyFcn=xlBlockMoveCallback(gcbh);  DeleteFcn=xlDestroyGui(gcbh);  ModelCloseFcn=xlDestroyGui(gcbh);  PreSaveFcn=xlBlockPreSaveCallback(gcbh);  PostSaveFcn=xlBlockPostSaveCallback(gcbh);  DestroyFcn=xlDestroyGui(gcbh);  OpenFcn=xlOpenGui(gcbh, 'negate_gui.xml', @negateenablement, -1)  CloseFcn=xlDestroyGui(gcbh);  MoveFcn=xlBlockMoveCallback(gcbh);
      mask Help: eval('');xlDoc('-book','sysgen','-topic','Negate');
      mask StyleString: edit,popup(Full|User Defined),edit,popup(Signed  (2's comp)|Unsigned),edit,edit,edit,popup(Truncate|Round  (unbiased: +/- Inf)),edit,popup(Wrap|Saturate|Flag as error),edit,checkbox,edit,edit,checkbox,edit,checkbox,edit,edit,edit,edit,edit,edit,edit,edit,edit
      mask Display:
      | fprintf('','COMMENT: begin icon graphics');
      | patch([0 55 55 0 0 ],[0 0 56 56 0 ],[0.77 0.82 0.91 ]);
      | plot([0 55 55 0 0 ],[0 0 56 56 0 ]);
      | patch([11.425 21.54 28.54 35.54 42.54 28.54 18.425 11.425 ],[35.77 35.77 42.77 35.77 42.77 42.77 42.77 35.77 ],[1 1 1 ]);
      | patch([18.425 28.54 21.54 11.425 18.425 ],[28.77 28.77 35.77 35.77 28.77 ],[0.931 0.946 0.973 ]);
      | patch([11.425 21.54 28.54 18.425 11.425 ],[21.77 21.77 28.77 28.77 21.77 ],[1 1 1 ]);
      | patch([18.425 42.54 35.54 28.54 21.54 11.425 18.425 ],[14.77 14.77 21.77 14.77 21.77 21.77 14.77 ],[0.931 0.946 0.973 ]);
      | fprintf('','COMMENT: end icon graphics');
      | fprintf('','COMMENT: begin icon text');
      | 
      | 
      | color('black');disp('\bf{x(-1)}','texmode','on');
      | fprintf('','COMMENT: end icon text');
  Opmode : S-Function  LoadFcn=xlBlockLoadCallback(gcbh);  FunctionName=sysgen  Parameters=ptable_  EnableBusSupport=off  mask(Xilinx Instruction Block Block){device_sgadvanced=, device=DSP48E, equ=P=C, operation_sgadvanced=, operation=C, inmode_0_3_sgadvanced=, inmode_0_3=D+A2, inmode_4_sgadvanced=, inmode_4=B2, logicinstr_sgadvanced=, logicinstr=X + Z, z_mux_sgadvanced=, z_mux=PCIN>>17, operand_sgadvanced=, operand=+, xy_mux_sgadvanced=, xy_mux=P, x_mux_sgadvanced=, x_mux=P, carry_sgadvanced=, carry=CIN, dbl_ovrd_sgadvanced=, dbl_ovrd=off, has_advanced_control=0, sggui_pos=-1,-1,-1,-1, block_type=opmode, block_version=, sg_icon_stat=55,26,0,1,white,blue,0,b91ab50c,right,,[ ],[ ], sg_mask_display=|, sg_list_contents=, sg_blockgui_xml=}
      mask sg_mask_display=|
      | fprintf('','COMMENT: begin icon graphics');
      | patch([0 55 55 0 0 ],[0 0 26 26 0 ],[0.77 0.82 0.91 ]);
      | plot([0 55 55 0 0 ],[0 0 26 26 0 ]);
      | patch([20.325 24.66 27.66 30.66 33.66 27.66 23.325 20.325 ],[16.33 16.33 19.33 16.33 19.33 19.33 19.33 16.33 ],[1 1 1 ]);
      | patch([23.325 27.66 24.66 20.325 23.325 ],[13.33 13.33 16.33 16.33 13.33 ],[0.931 0.946 0.973 ]);
      | patch([20.325 24.66 27.66 23.325 20.325 ],[10.33 10.33 13.33 13.33 10.33 ],[1 1 1 ]);
      | patch([23.325 33.66 30.66 27.66 24.66 20.325 23.325 ],[7.33 7.33 10.33 7.33 10.33 10.33 7.33 ],[0.931 0.946 0.973 ]);
      | fprintf('','COMMENT: end icon graphics');
      | fprintf('','COMMENT: begin icon text');
      | color('black');port_label('output',1,'P=C');
      | fprintf('','COMMENT: end icon text');
      mask prompts: device_sgadvanced ""; equ "Operation"; operation_sgadvanced ""; operation "Operation select"; inmode_0_3_sgadvanced ""; inmode_0_3 "Preadder output"; inmode_4_sgadvanced ""; inmode_4 "<tt>B</tt> register configuration"; logicinstr_sgadvanced ""; logicinstr "Instruction"; z_mux_sgadvanced ""; z_mux "Z mux"; operand_sgadvanced ""; xy_mux_sgadvanced ""; xy_mux "XY muxes"; x_mux_sgadvanced ""; x_mux "X mux"; carry_sgadvanced ""; carry "Carry input"; dbl_ovrd_sgadvanced ""; dbl_ovrd "Override with doubles"; has_advanced_control ""; sggui_pos ""; block_type ""; block_version ""; sg_icon_stat ""; sg_mask_display ""; sg_list_contents ""; sg_blockgui_xml ""
      mask help: Xilinx Instruction Block
      mask init:
      | try
      |   tmp_gcb = gcb;
      |   tmp_gcbh = gcbh;
      |   if (strcmp('SysGenIndex',get_param(bdroot(tmp_gcbh),'tag')) && ~isempty(regexp(bdroot(tmp_gcb), '^xbs', 'once')))
      |     return;
      |   end;
      |   xlMungeMaskParams;
      |   block_config = 'sysgen_blockset:Opmode_config';
      | 
      |   block_type='opmode';
      | 
      |   serialized_declarations = '{''carry''=>''String'',''dbl_ovrd''=>''Int'',''device''=>''Int'',''equ''=>''String'',''inmode_0_3''=>''String'',''inmode_4''=>''Int'',''logicinstr''=>''Int'',''operand''=>''Int'',''operation''=>''String'',''x_mux''=>''Int'',''xy_mux''=>''Int'',''z_mux''=>''String'',''block_type''=>''String''}';
      |   ptable_ = xlblockprep(get_param(tmp_gcb, 'MaskWSVariables'));
      |   try
      |     xlBlockMoveCallback(tmp_gcbh);
      |   catch 
      |      clear global xl_updateicon_recursion_guard;
      |   end;
      | catch
      |   global dbgsysgen;
      |   if(~isempty(dbgsysgen) && dbgsysgen)
      |     e = regexprep(lasterr, '\n', '\nError: ');
      |     disp(['Error: While running MaskInit code on block ' tmp_gcb ': ' e]);
      |     error(e);
      |   end
      | end
      settings: CopyFcn=xlBlockMoveCallback(gcbh);  DeleteFcn=xlDestroyGui(gcbh);  ModelCloseFcn=xlDestroyGui(gcbh);  PreSaveFcn=xlBlockPreSaveCallback(gcbh);  PostSaveFcn=xlBlockPostSaveCallback(gcbh);  DestroyFcn=xlDestroyGui(gcbh);  OpenFcn=xlOpenGui(gcbh, 'opmode_gui.xml', @opmodeenablement, @opmodeaction)  CloseFcn=xlDestroyGui(gcbh);  MoveFcn=xlBlockMoveCallback(gcbh);
      mask Help: eval('');xlDoc('-book','sysgen','-topic','Opmode');
      mask StyleString: edit,popup(DSP48E1|DSP48E|DSP48|DSP48A),edit,edit,popup(C + A*B|PCIN + A*B|P + A*B|A * B|C + A:B|C - A:B|C|Custom|C + D:A:B|C - D:A:B),edit,popup(Zero|A2|A1|D+A2|D+A1|D|-A2|-A1|D-A2|D-A1),edit,popup(B1|B2),edit,popup(X + Z|X + NOT(Z)|NOT(X + Z)|Z - X|X XOR Z|X XNOR Z|X AND Z|X OR Z|X AND NOT(Z)|X OR NOT(Z)|X NAND Z|X NOR Z|NOT(X) OR Z|NOT(X) AND Z),edit,popup(0|PCIN|P|C|PCIN>>17|P>>17),edit,popup(+|-),edit,popup(0|P|A:B|A*B|C|P+C|A:B+C),edit,popup(0|P|A*B|A*(D+B)|A*(D-B)|D:A:B|D:A:(D+B)|D:A:(D-B)),edit,popup(0|1|CIN|Round PCIN towards infinity|Round PCIN towards zero|Round P towards infinity|Round P towards zero|Larger add/sub/acc (parallel operation)|Larger add/sub/acc (sequential operation)|Round A*B),edit,checkbox,edit,edit,edit,edit,edit,edit,edit,edit
      mask Display:
      | fprintf('','COMMENT: begin icon graphics');
      | patch([0 55 55 0 0 ],[0 0 26 26 0 ],[0.77 0.82 0.91 ]);
      | plot([0 55 55 0 0 ],[0 0 26 26 0 ]);
      | patch([20.325 24.66 27.66 30.66 33.66 27.66 23.325 20.325 ],[16.33 16.33 19.33 16.33 19.33 19.33 19.33 16.33 ],[1 1 1 ]);
      | patch([23.325 27.66 24.66 20.325 23.325 ],[13.33 13.33 16.33 16.33 13.33 ],[0.931 0.946 0.973 ]);
      | patch([20.325 24.66 27.66 23.325 20.325 ],[10.33 10.33 13.33 13.33 10.33 ],[1 1 1 ]);
      | patch([23.325 33.66 30.66 27.66 24.66 20.325 23.325 ],[7.33 7.33 10.33 7.33 10.33 10.33 7.33 ],[0.931 0.946 0.973 ]);
      | fprintf('','COMMENT: end icon graphics');
      | fprintf('','COMMENT: begin icon text');
      | color('black');port_label('output',1,'P=C');
      | fprintf('','COMMENT: end icon text');
  Parallel to Serial : S-Function  LoadFcn=xlBlockLoadCallback(gcbh);  FunctionName=sysgen  Parameters=ptable_  EnableBusSupport=off  mask(Xilinx Parallel to Serial Converter Block){infoedit=Each sample presented at the input becomes several samples presented serially at the output., output_order_sgadvanced=, output_order=Least Significant Word First, arith_type_sgadvanced=, arith_type=Unsigned, output_bits=1, bin_pt=0, rst_sgadvanced=, rst=off, en_sgadvanced=, en=off, latency=0, dbl_ovrd_sgadvanced=, dbl_ovrd=off, xl_use_area_sgadvanced=, xl_use_area=off, xl_area=[0,0,0,0,0,0,0], has_advanced_control=0, sggui_pos=-1,-1,-1,-1, block_type=p2s, block_version=, sg_icon_stat=55,58,1,1,white,blue,0,020e968f,right,,[ ],[ ], sg_mask_display=|, sg_list_contents=, sg_blockgui_xml=}
      mask sg_mask_display=|
      | fprintf('','COMMENT: begin icon graphics');
      | patch([0 55 55 0 0 ],[0 0 58 58 0 ],[0.77 0.82 0.91 ]);
      | plot([0 55 55 0 0 ],[0 0 58 58 0 ]);
      | patch([11.425 21.54 28.54 35.54 42.54 28.54 18.425 11.425 ],[36.77 36.77 43.77 36.77 43.77 43.77 43.77 36.77 ],[1 1 1 ]);
      | patch([18.425 28.54 21.54 11.425 18.425 ],[29.77 29.77 36.77 36.77 29.77 ],[0.931 0.946 0.973 ]);
      | patch([11.425 21.54 28.54 18.425 11.425 ],[22.77 22.77 29.77 29.77 22.77 ],[1 1 1 ]);
      | patch([18.425 42.54 35.54 28.54 21.54 11.425 18.425 ],[15.77 15.77 22.77 15.77 22.77 22.77 15.77 ],[0.931 0.946 0.973 ]);
      | fprintf('','COMMENT: end icon graphics');
      | fprintf('','COMMENT: begin icon text');
      | color('black');port_label('input',1,'p');
      | color('black');port_label('output',1,'s');
      | fprintf('','COMMENT: end icon text');
      mask prompts: infoedit ""; output_order_sgadvanced ""; output_order "Output order"; arith_type_sgadvanced ""; arith_type "Type"; output_bits "Number of bits"; bin_pt "Binary point"; rst_sgadvanced ""; rst "Provide <tt>reset</tt> port"; en_sgadvanced ""; en "Provide <tt>enable</tt> port"; dbl_ovrd_sgadvanced ""; dbl_ovrd "Override with doubles"; xl_use_area_sgadvanced ""; xl_use_area "Define FPGA area for resource estimation"; xl_area "FPGA area [slices, FFs, BRAMs, LUTs, IOBs, emb. mults, TBUFs]"; has_advanced_control ""; sggui_pos ""; block_type ""; block_version ""; sg_icon_stat ""; sg_mask_display ""; sg_list_contents ""; sg_blockgui_xml ""
      mask help: Each sample presented at the input becomes several samples presented serially at the output.
      mask init:
      | try
      |   tmp_gcb = gcb;
      |   tmp_gcbh = gcbh;
      |   if (strcmp('SysGenIndex',get_param(bdroot(tmp_gcbh),'tag')) && ~isempty(regexp(bdroot(tmp_gcb), '^xbs', 'once')))
      |     return;
      |   end;
      |   xlMungeMaskParams;
      |   block_config = 'sysgen_blockset:P2S_config';
      | 
      |   block_type='p2s';
      | 
      |   serialized_declarations = '{''arith_type''=>''Int'',''bin_pt''=>''Int'',''dbl_ovrd''=>''Int'',''en''=>''Int'',''latency''=>''Int'',''output_bits''=>''Int'',''output_order''=>''Int'',''rst''=>''Bool'',''sim_engine''=>''Int'',''sysgen_root''=>''String'',''block_type''=>''String''}';
      |   xlp2s_init();
      |   ptable_ = xlblockprep(get_param(tmp_gcb, 'MaskWSVariables'));
      |   try
      |     xlBlockMoveCallback(tmp_gcbh);
      |   catch 
      |      clear global xl_updateicon_recursion_guard;
      |   end;
      | catch
      |   global dbgsysgen;
      |   if(~isempty(dbgsysgen) && dbgsysgen)
      |     e = regexprep(lasterr, '\n', '\nError: ');
      |     disp(['Error: While running MaskInit code on block ' tmp_gcb ': ' e]);
      |     error(e);
      |   end
      | end
      settings: CopyFcn=xlBlockMoveCallback(gcbh);  DeleteFcn=xlDestroyGui(gcbh);  ModelCloseFcn=xlDestroyGui(gcbh);  PreSaveFcn=xlBlockPreSaveCallback(gcbh);  PostSaveFcn=xlBlockPostSaveCallback(gcbh);  DestroyFcn=xlDestroyGui(gcbh);  OpenFcn=xlOpenGui(gcbh, 'p2s_gui.xml', @xlmagicenablement, -1)  CloseFcn=xlDestroyGui(gcbh);  MoveFcn=xlBlockMoveCallback(gcbh);
      mask Help: eval('');xlDoc('-book','sysgen','-topic','Parallel_to_Serial');
      mask StyleString: edit,edit,popup(Least Significant Word First|Most Significant Word First),edit,popup(Signed  (2's comp)|Unsigned),edit,edit,edit,checkbox,edit,checkbox,edit,edit,checkbox,edit,checkbox,edit,edit,edit,edit,edit,edit,edit,edit,edit
      mask Display:
      | fprintf('','COMMENT: begin icon graphics');
      | patch([0 55 55 0 0 ],[0 0 58 58 0 ],[0.77 0.82 0.91 ]);
      | plot([0 55 55 0 0 ],[0 0 58 58 0 ]);
      | patch([11.425 21.54 28.54 35.54 42.54 28.54 18.425 11.425 ],[36.77 36.77 43.77 36.77 43.77 43.77 43.77 36.77 ],[1 1 1 ]);
      | patch([18.425 28.54 21.54 11.425 18.425 ],[29.77 29.77 36.77 36.77 29.77 ],[0.931 0.946 0.973 ]);
      | patch([11.425 21.54 28.54 18.425 11.425 ],[22.77 22.77 29.77 29.77 22.77 ],[1 1 1 ]);
      | patch([18.425 42.54 35.54 28.54 21.54 11.425 18.425 ],[15.77 15.77 22.77 15.77 22.77 22.77 15.77 ],[0.931 0.946 0.973 ]);
      | fprintf('','COMMENT: end icon graphics');
      | fprintf('','COMMENT: begin icon text');
      | color('black');port_label('input',1,'p');
      | color('black');port_label('output',1,'s');
      | fprintf('','COMMENT: end icon text');
  Pause Simulation : Subsystem  LoadFcn=xlBlockLoadCallback(gcbh);  mask(Xilinx Pause Simulation. Block){infoedit=Pause simulation.  Pauses simulation when input is nonzero., has_advanced_control=0, sggui_pos=-1,-1,-1,-1, block_type=pausesim, block_version=, sg_icon_stat=55,48,-1,-1,blue,white,0,07734,right,,[ ],[ ], sg_mask_display=|, sg_list_contents=, sg_blockgui_xml=}
      mask sg_mask_display=|
      | fprintf('','COMMENT: begin icon graphics');
      | patch([0 55 55 0 0 ],[0 0 48 48 0 ],[1 1 1 ]);
      | plot([0 55 55 0 0 ],[0 0 48 48 0 ]);
      | patch([13.65 22.32 28.32 34.32 40.32 28.32 19.65 13.65 ],[30.66 30.66 36.66 30.66 36.66 36.66 36.66 30.66 ],[0.839 0.874 0.937 ]);
      | patch([19.65 28.32 22.32 13.65 19.65 ],[24.66 24.66 30.66 30.66 24.66 ],[0.77 0.82 0.91 ]);
      | patch([13.65 22.32 28.32 19.65 13.65 ],[18.66 18.66 24.66 24.66 18.66 ],[0.839 0.874 0.937 ]);
      | patch([19.65 40.32 34.32 28.32 22.32 13.65 19.65 ],[12.66 12.66 18.66 12.66 18.66 18.66 12.66 ],[0.77 0.82 0.91 ]);
      | fprintf('','COMMENT: end icon graphics');
      | fprintf('','COMMENT: begin icon text');
      | fprintf('','COMMENT: end icon text');
      mask prompts: infoedit ""; has_advanced_control ""; sggui_pos ""; block_type ""; block_version ""; sg_icon_stat ""; sg_mask_display ""; sg_list_contents ""; sg_blockgui_xml ""
      mask help: Pause simulation. Pauses simulation when input is nonzero.
      mask init:
      | try
      |   tmp_gcb = gcb;
      |   tmp_gcbh = gcbh;
      |   if (strcmp('SysGenIndex',get_param(bdroot(tmp_gcbh),'tag')) && ~isempty(regexp(bdroot(tmp_gcb), '^xbs', 'once')))
      |     return;
      |   end;
      |   xlMungeMaskParams;
      | 
      |   block_type='pausesim';
      | 
      |   serialized_declarations = '{''block_type''=>''String''}';
      |   xlpausesim_init();
      |   ptable_ = xlblockprep(get_param(tmp_gcb, 'MaskWSVariables'));
      |   try
      |     xlBlockMoveCallback(tmp_gcbh);
      |   catch 
      |      clear global xl_updateicon_recursion_guard;
      |   end;
      | catch
      |   global dbgsysgen;
      |   if(~isempty(dbgsysgen) && dbgsysgen)
      |     e = regexprep(lasterr, '\n', '\nError: ');
      |     disp(['Error: While running MaskInit code on block ' tmp_gcb ': ' e]);
      |     error(e);
      |   end
      | end
      settings: CopyFcn=xlBlockMoveCallback(gcbh);  DeleteFcn=xlDestroyGui(gcbh);  ModelCloseFcn=xlDestroyGui(gcbh);  PreSaveFcn=xlBlockPreSaveCallback(gcbh);  PostSaveFcn=xlBlockPostSaveCallback(gcbh);  DestroyFcn=xlDestroyGui(gcbh);  OpenFcn=xlOpenGui(gcbh, 'pausesim_gui.xml', -1, -1)  CloseFcn=xlDestroyGui(gcbh);  MoveFcn=xlBlockMoveCallback(gcbh);
      mask Help: eval('');xlDoc('-book','sysgen','-topic','Pause_Simulation');
      mask Display:
      | fprintf('','COMMENT: begin icon graphics');
      | patch([0 55 55 0 0 ],[0 0 48 48 0 ],[1 1 1 ]);
      | plot([0 55 55 0 0 ],[0 0 48 48 0 ]);
      | patch([13.65 22.32 28.32 34.32 40.32 28.32 19.65 13.65 ],[30.66 30.66 36.66 30.66 36.66 36.66 36.66 30.66 ],[0.839 0.874 0.937 ]);
      | patch([19.65 28.32 22.32 13.65 19.65 ],[24.66 24.66 30.66 30.66 24.66 ],[0.77 0.82 0.91 ]);
      | patch([13.65 22.32 28.32 19.65 13.65 ],[18.66 18.66 24.66 24.66 18.66 ],[0.839 0.874 0.937 ]);
      | patch([19.65 40.32 34.32 28.32 22.32 13.65 19.65 ],[12.66 12.66 18.66 12.66 18.66 18.66 12.66 ],[0.77 0.82 0.91 ]);
      | fprintf('','COMMENT: end icon graphics');
      | fprintf('','COMMENT: begin icon text');
      | fprintf('','COMMENT: end icon text');
  PicoBlaze Microcontroller : S-Function  LoadFcn=xlBlockLoadCallback(gcbh);  FunctionName=sysgen  Parameters=ptable_  EnableBusSupport=off  mask(Xilinx PicoBlaze Microcontroller Block){version_sgadvanced=, version=PicoBlaze 2, display_mi_sgadvanced=, display_mi=off, xl_view_as_sgadvanced=, xl_view_as=Decimal, xl_use_area_sgadvanced=, xl_use_area=off, xl_area=[0,0,0,0,0,0,0], has_advanced_control=0, sggui_pos=-1,-1,-1,-1, block_type=pb, block_version=, sg_icon_stat=95,78,4,5,white,blue,0,62087863,right,,[ ],[ ], sg_mask_display=|, sg_list_contents=, sg_blockgui_xml=}
      mask sg_mask_display=|
      | fprintf('','COMMENT: begin icon graphics');
      | patch([0 95 95 0 0 ],[0 0 78 78 0 ],[0.77 0.82 0.91 ]);
      | plot([0 95 95 0 0 ],[0 0 78 78 0 ]);
      | patch([22.525 38.42 49.42 60.42 71.42 49.42 33.525 22.525 ],[51.21 51.21 62.21 51.21 62.21 62.21 62.21 51.21 ],[1 1 1 ]);
      | patch([33.525 49.42 38.42 22.525 33.525 ],[40.21 40.21 51.21 51.21 40.21 ],[0.931 0.946 0.973 ]);
      | patch([22.525 38.42 49.42 33.525 22.525 ],[29.21 29.21 40.21 40.21 29.21 ],[1 1 1 ]);
      | patch([33.525 71.42 60.42 49.42 38.42 22.525 33.525 ],[18.21 18.21 29.21 18.21 29.21 29.21 18.21 ],[0.931 0.946 0.973 ]);
      | fprintf('','COMMENT: end icon graphics');
      | fprintf('','COMMENT: begin icon text');
      | color('black');port_label('input',1,'in_port');
      | color('black');port_label('input',2,'brk');
      | color('black');port_label('input',3,'rst');
      | color('black');port_label('input',4,'instr');
      | color('black');port_label('output',1,'out_port');
      | color('black');port_label('output',2,'port_id');
      | color('black');port_label('output',3,'rs');
      | color('black');port_label('output',4,'ws');
      | color('black');port_label('output',5,'addr');
      | fprintf('','COMMENT: end icon text');
      mask prompts: version_sgadvanced ""; display_mi_sgadvanced ""; display_mi "Display internal state"; xl_view_as_sgadvanced ""; xl_view_as "Display values as"; xl_use_area_sgadvanced ""; xl_use_area "Define FPGA area for resource estimation"; xl_area "FPGA area [slices, FFs, BRAMs, LUTs, IOBs, emb. mults, TBUFs]"; has_advanced_control ""; sggui_pos ""; block_type ""; block_version ""; sg_icon_stat ""; sg_mask_display ""; sg_list_contents ""; sg_blockgui_xml ""
      mask help: Xilinx PicoBlaze Microcontroller
      mask init:
      | try
      |   tmp_gcb = gcb;
      |   tmp_gcbh = gcbh;
      |   if (strcmp('SysGenIndex',get_param(bdroot(tmp_gcbh),'tag')) && ~isempty(regexp(bdroot(tmp_gcb), '^xbs', 'once')))
      |     return;
      |   end;
      |   xlMungeMaskParams;
      |   block_config = 'sysgen_blockset:PicoBlaze_config';
      | 
      |   block_type='pb';
      | 
      |   serialized_declarations = '{''debug_mode''=>''Int'',''period''=>''Double'',''program_file''=>''String'',''version''=>''Int'',''xl_view_as''=>''Int'',''block_type''=>''String''}';
      |   xlpb_init();
      |   ptable_ = xlblockprep(get_param(tmp_gcb, 'MaskWSVariables'));
      |   try
      |     xlBlockMoveCallback(tmp_gcbh);
      |   catch 
      |      clear global xl_updateicon_recursion_guard;
      |   end;
      | catch
      |   global dbgsysgen;
      |   if(~isempty(dbgsysgen) && dbgsysgen)
      |     e = regexprep(lasterr, '\n', '\nError: ');
      |     disp(['Error: While running MaskInit code on block ' tmp_gcb ': ' e]);
      |     error(e);
      |   end
      | end
      settings: CopyFcn=xlBlockMoveCallback(gcbh);  DeleteFcn=xlDestroyGui(gcbh);  ModelCloseFcn=xlDestroyGui(gcbh);  PreSaveFcn=xlBlockPreSaveCallback(gcbh);  PostSaveFcn=xlBlockPostSaveCallback(gcbh);  DestroyFcn=xlDestroyGui(gcbh);  OpenFcn=xlOpenGui(gcbh, 'pb_gui.xml', @pbenablement, -1)  CloseFcn=xlDestroyGui(gcbh);  MoveFcn=xlBlockMoveCallback(gcbh);
      mask Help: eval('');xlDoc('-book','sysgen','-topic','PicoBlaze_Microcontroller');
      mask StyleString: edit,popup(PicoBlaze 2|PicoBlaze 3),edit,checkbox,edit,popup(Decimal|Hexadecimal),edit,checkbox,edit,edit,edit,edit,edit,edit,edit,edit,edit
      mask Display:
      | fprintf('','COMMENT: begin icon graphics');
      | patch([0 95 95 0 0 ],[0 0 78 78 0 ],[0.77 0.82 0.91 ]);
      | plot([0 95 95 0 0 ],[0 0 78 78 0 ]);
      | patch([22.525 38.42 49.42 60.42 71.42 49.42 33.525 22.525 ],[51.21 51.21 62.21 51.21 62.21 62.21 62.21 51.21 ],[1 1 1 ]);
      | patch([33.525 49.42 38.42 22.525 33.525 ],[40.21 40.21 51.21 51.21 40.21 ],[0.931 0.946 0.973 ]);
      | patch([22.525 38.42 49.42 33.525 22.525 ],[29.21 29.21 40.21 40.21 29.21 ],[1 1 1 ]);
      | patch([33.525 71.42 60.42 49.42 38.42 22.525 33.525 ],[18.21 18.21 29.21 18.21 29.21 29.21 18.21 ],[0.931 0.946 0.973 ]);
      | fprintf('','COMMENT: end icon graphics');
      | fprintf('','COMMENT: begin icon text');
      | color('black');port_label('input',1,'in_port');
      | color('black');port_label('input',2,'brk');
      | color('black');port_label('input',3,'rst');
      | color('black');port_label('input',4,'instr');
      | color('black');port_label('output',1,'out_port');
      | color('black');port_label('output',2,'port_id');
      | color('black');port_label('output',3,'rs');
      | color('black');port_label('output',4,'ws');
      | color('black');port_label('output',5,'addr');
      | fprintf('','COMMENT: end icon text');
  PicoBlaze Instruction Display : Subsystem  LoadFcn=global xl_pb_trace;  mask(Xilinx PicoBlaze Microcontroller Instruction Display Block){infoedit=PicoBlaze Instruction\nDisplay, xl_pb_inst=LOAD s6, s7, xl_pb_pc=28, xl_pb_version_sgadvanced=, xl_pb_version=Must Specify, xl_pb_disable_sgadvanced=, xl_pb_disable=off, has_advanced_control=0, sggui_pos=-1,-1,-1,-1, block_type=picoblaze_instruction_display, block_version=, sg_icon_stat=95,80,-1,-1,blue,white,0,07734,right,,[ ],[ ], sg_mask_display=|, sg_list_contents=, sg_blockgui_xml=}
      mask sg_mask_display=|
      | fprintf('','COMMENT: begin icon graphics');
      | patch([0 95 95 0 0 ],[0 0 80 80 0 ],[1 1 1 ]);
      | plot([0 95 95 0 0 ],[0 0 80 80 0 ]);
      | patch([22.525 38.42 49.42 60.42 71.42 49.42 33.525 22.525 ],[52.21 52.21 63.21 52.21 63.21 63.21 63.21 52.21 ],[0.839 0.874 0.937 ]);
      | patch([33.525 49.42 38.42 22.525 33.525 ],[41.21 41.21 52.21 52.21 41.21 ],[0.77 0.82 0.91 ]);
      | patch([22.525 38.42 49.42 33.525 22.525 ],[30.21 30.21 41.21 41.21 30.21 ],[0.839 0.874 0.937 ]);
      | patch([33.525 71.42 60.42 49.42 38.42 22.525 33.525 ],[19.21 19.21 30.21 19.21 30.21 30.21 19.21 ],[0.77 0.82 0.91 ]);
      | fprintf('','COMMENT: end icon graphics');
      | fprintf('','COMMENT: begin icon text');
      | fprintf('','COMMENT: end icon text');fprintf('Inst: %s\nProgCnt: %d', xl_pb_inst, xl_pb_pc);
      | port_label('input',1,'instr');
      | port_label('input',2,'addr');
      mask prompts: infoedit ""; xl_pb_inst ""; xl_pb_pc ""; xl_pb_version_sgadvanced ""; xl_pb_version "Version"; xl_pb_disable_sgadvanced ""; xl_pb_disable "Disable Display"; has_advanced_control ""; sggui_pos ""; block_type ""; block_version ""; sg_icon_stat ""; sg_mask_display ""; sg_list_contents ""; sg_blockgui_xml ""
      mask help: PicoBlaze Instruction\nDisplay
      mask init:
      | try
      |   tmp_gcb = gcb;
      |   tmp_gcbh = gcbh;
      |   if (strcmp('SysGenIndex',get_param(bdroot(tmp_gcbh),'tag')) && ~isempty(regexp(bdroot(tmp_gcb), '^xbs', 'once')))
      |     return;
      |   end;
      |   xlMungeMaskParams;
      | 
      |   block_type='picoblaze_instruction_display';
      | 
      |   serialized_declarations = '{''block_type''=>''String''}';
      |   ptable_ = xlblockprep(get_param(tmp_gcb, 'MaskWSVariables'));
      |   try
      |     xlBlockMoveCallback(tmp_gcbh);
      |   catch 
      |      clear global xl_updateicon_recursion_guard;
      |   end;
      | catch
      |   global dbgsysgen;
      |   if(~isempty(dbgsysgen) && dbgsysgen)
      |     e = regexprep(lasterr, '\n', '\nError: ');
      |     disp(['Error: While running MaskInit code on block ' tmp_gcb ': ' e]);
      |     error(e);
      |   end
      | end
      settings: CopyFcn=xlBlockMoveCallback(gcbh);  MoveFcn=xlBlockMoveCallback(gcbh);
      mask Help: eval('');xlDoc('-book','sysgen','-topic','PicoBlaze_Instruction_Display');
      mask StyleString: edit,edit,edit,edit,popup(Must Specify|PicoBlaze 2|PicoBlaze 3),edit,checkbox,edit,edit,edit,edit,edit,edit,edit,edit
      mask Display:
      | fprintf('','COMMENT: begin icon graphics');
      | patch([0 95 95 0 0 ],[0 0 80 80 0 ],[1 1 1 ]);
      | plot([0 95 95 0 0 ],[0 0 80 80 0 ]);
      | patch([22.525 38.42 49.42 60.42 71.42 49.42 33.525 22.525 ],[52.21 52.21 63.21 52.21 63.21 63.21 63.21 52.21 ],[0.839 0.874 0.937 ]);
      | patch([33.525 49.42 38.42 22.525 33.525 ],[41.21 41.21 52.21 52.21 41.21 ],[0.77 0.82 0.91 ]);
      | patch([22.525 38.42 49.42 33.525 22.525 ],[30.21 30.21 41.21 41.21 30.21 ],[0.839 0.874 0.937 ]);
      | patch([33.525 71.42 60.42 49.42 38.42 22.525 33.525 ],[19.21 19.21 30.21 19.21 30.21 30.21 19.21 ],[0.77 0.82 0.91 ]);
      | fprintf('','COMMENT: end icon graphics');
      | fprintf('','COMMENT: begin icon text');
      | fprintf('','COMMENT: end icon text');fprintf('Inst: %s\nProgCnt: %d', xl_pb_inst, xl_pb_pc);
      | port_label('input',1,'instr');
      | port_label('input',2,'addr');
  Puncture : S-Function  LoadFcn=xlBlockLoadCallback(gcbh);  FunctionName=sysgen  Parameters=ptable_  EnableBusSupport=off  mask(Xilinx Puncturer Block){infoedit=Reads values from the input port, removes the bits corresponding to zeros in the puncture code, then presents the remaining bits at the output port.<br><br>Hardware notes: In hardware this block costs nothing., punc_char=[1 0 0], dbl_ovrd_sgadvanced=, dbl_ovrd=off, has_advanced_control=0, sggui_pos=-1,-1,-1,-1, block_type=puncture, block_version=, sg_icon_stat=55,32,1,1,white,blue,0,d8a4170d,right,,[ ],[ ], sg_mask_display=|, sg_list_contents=, sg_blockgui_xml=}
      mask sg_mask_display=|
      | fprintf('','COMMENT: begin icon graphics');
      | patch([0 55 55 0 0 ],[0 0 32 32 0 ],[0.77 0.82 0.91 ]);
      | plot([0 55 55 0 0 ],[0 0 32 32 0 ]);
      | patch([18.1 23.88 27.88 31.88 35.88 27.88 22.1 18.1 ],[20.44 20.44 24.44 20.44 24.44 24.44 24.44 20.44 ],[1 1 1 ]);
      | patch([22.1 27.88 23.88 18.1 22.1 ],[16.44 16.44 20.44 20.44 16.44 ],[0.931 0.946 0.973 ]);
      | patch([18.1 23.88 27.88 22.1 18.1 ],[12.44 12.44 16.44 16.44 12.44 ],[1 1 1 ]);
      | patch([22.1 35.88 31.88 27.88 23.88 18.1 22.1 ],[8.44 8.44 12.44 8.44 12.44 12.44 8.44 ],[0.931 0.946 0.973 ]);
      | fprintf('','COMMENT: end icon graphics');
      | fprintf('','COMMENT: begin icon text');
      |
      |
      | color('black');disp('Puncture');
      | fprintf('','COMMENT: end icon text');
      mask prompts: infoedit ""; punc_char "Puncture code"; dbl_ovrd_sgadvanced ""; dbl_ovrd "Override with doubles"; has_advanced_control ""; sggui_pos ""; block_type ""; block_version ""; sg_icon_stat ""; sg_mask_display ""; sg_list_contents ""; sg_blockgui_xml ""
      mask help:
      | Reads values from the input port, removes the bits corresponding to zeros in the puncture code, then presents the remaining bits at the output port.
      |
      | Hardware notes: In hardware this block costs nothing.
      mask init:
      | try
      |   tmp_gcb = gcb;
      |   tmp_gcbh = gcbh;
      |   if (strcmp('SysGenIndex',get_param(bdroot(tmp_gcbh),'tag')) && ~isempty(regexp(bdroot(tmp_gcb), '^xbs', 'once')))
      |     return;
      |   end;
      |   xlMungeMaskParams;
      |   block_config = 'sysgen_blockset:Puncture_config';
      | 
      |   block_type='puncture';
      | 
      |   serialized_declarations = '{''punc_char''=>''IntVector'',''block_type''=>''String''}';
      |   ptable_ = xlblockprep(get_param(tmp_gcb, 'MaskWSVariables'));
      |   try
      |     xlBlockMoveCallback(tmp_gcbh);
      |   catch 
      |      clear global xl_updateicon_recursion_guard;
      |   end;
      | catch
      |   global dbgsysgen;
      |   if(~isempty(dbgsysgen) && dbgsysgen)
      |     e = regexprep(lasterr, '\n', '\nError: ');
      |     disp(['Error: While running MaskInit code on block ' tmp_gcb ': ' e]);
      |     error(e);
      |   end
      | end
      settings: CopyFcn=xlBlockMoveCallback(gcbh);  DeleteFcn=xlDestroyGui(gcbh);  ModelCloseFcn=xlDestroyGui(gcbh);  PreSaveFcn=xlBlockPreSaveCallback(gcbh);  PostSaveFcn=xlBlockPostSaveCallback(gcbh);  DestroyFcn=xlDestroyGui(gcbh);  OpenFcn=xlOpenGui(gcbh, 'puncture_gui.xml', @xlmagicenablement, -1)  CloseFcn=xlDestroyGui(gcbh);  MoveFcn=xlBlockMoveCallback(gcbh);
      mask Help: eval('');xlDoc('-book','sysgen','-topic','Puncture');
      mask Display:
      | fprintf('','COMMENT: begin icon graphics');
      | patch([0 55 55 0 0 ],[0 0 32 32 0 ],[0.77 0.82 0.91 ]);
      | plot([0 55 55 0 0 ],[0 0 32 32 0 ]);
      | patch([18.1 23.88 27.88 31.88 35.88 27.88 22.1 18.1 ],[20.44 20.44 24.44 20.44 24.44 24.44 24.44 20.44 ],[1 1 1 ]);
      | patch([22.1 27.88 23.88 18.1 22.1 ],[16.44 16.44 20.44 20.44 16.44 ],[0.931 0.946 0.973 ]);
      | patch([18.1 23.88 27.88 22.1 18.1 ],[12.44 12.44 16.44 16.44 12.44 ],[1 1 1 ]);
      | patch([22.1 35.88 31.88 27.88 23.88 18.1 22.1 ],[8.44 8.44 12.44 8.44 12.44 12.44 8.44 ],[0.931 0.946 0.973 ]);
      | fprintf('','COMMENT: end icon graphics');
      | fprintf('','COMMENT: begin icon text');
      | 
      | 
      | color('black');disp('Puncture');
      | fprintf('','COMMENT: end icon text');
  ROM : S-Function  LoadFcn=xlBlockLoadCallback(gcbh);  FunctionName=sysgen  Parameters=ptable_  EnableBusSupport=off  mask(Xilinx Single Port Read-Only Memory Block){depth=16, initVector=sin(pi*(0:15)/16), distributed_mem_sgadvanced=, distributed_mem=Block RAM, rst_sgadvanced=, rst=off, init_reg=0, en_sgadvanced=, en=off, latency=1, gui_display_data_type_sgadvanced=, gui_display_data_type=Fixed-point, arith_type_sgadvanced=, arith_type=Signed  (2's comp), n_bits=16, bin_pt=14, preci_type_sgadvanced=, preci_type=Single, exp_width=8, frac_width=24, dbl_ovrd_sgadvanced=, dbl_ovrd=off, optimize_sgadvanced=, optimize=Area, use_rpm_sgadvanced=, use_rpm=on, xl_use_area_sgadvanced=, xl_use_area=off, xl_area=[0,0,0,0,0,0,0], has_advanced_control=0, sggui_pos=-1,-1,-1,-1, block_type=sprom, block_version=, sg_icon_stat=60,56,1,1,white,blue,0,bbc23d60,right,,[ ],[ ], sg_mask_display=|, sg_list_contents=, sg_blockgui_xml=}
      mask sg_mask_display=|
      | fprintf('','COMMENT: begin icon graphics');
      | patch([0 60 60 0 0 ],[0 0 56 56 0 ],[0.77 0.82 0.91 ]);
      | plot([0 60 60 0 0 ],[0 0 56 56 0 ]);
      | patch([12.2 23.76 31.76 39.76 47.76 31.76 20.2 12.2 ],[36.88 36.88 44.88 36.88 44.88 44.88 44.88 36.88 ],[1 1 1 ]);
      | patch([20.2 31.76 23.76 12.2 20.2 ],[28.88 28.88 36.88 36.88 28.88 ],[0.931 0.946 0.973 ]);
      | patch([12.2 23.76 31.76 20.2 12.2 ],[20.88 20.88 28.88 28.88 20.88 ],[1 1 1 ]);
      | patch([20.2 47.76 39.76 31.76 23.76 12.2 20.2 ],[12.88 12.88 20.88 12.88 20.88 20.88 12.88 ],[0.931 0.946 0.973 ]);
      | fprintf('','COMMENT: end icon graphics');
      | fprintf('','COMMENT: begin icon text');
      | color('black');port_label('input',1,'addr');
      |
      | color('black');disp('z^{-1}','texmode','on');
      | fprintf('','COMMENT: end icon text');
      mask prompts: initVector "Initial value vector"; distributed_mem_sgadvanced ""; distributed_mem "Memory Type"; rst_sgadvanced ""; rst "Provide reset port for output register"; init_reg "Initial value for output register"; en_sgadvanced ""; en "Provide enable port"; gui_display_data_type_sgadvanced ""; gui_display_data_type ""; arith_type_sgadvanced ""; arith_type "Arithmetic type"; n_bits "Number of bits"; bin_pt "Binary point"; preci_type_sgadvanced ""; preci_type ""; exp_width "Exponent width"; frac_width "Fraction width"; dbl_ovrd_sgadvanced ""; dbl_ovrd "Override with doubles"; optimize_sgadvanced ""; optimize "Optimize for"; use_rpm_sgadvanced ""; use_rpm "Use pre-defined core placement information"; xl_use_area_sgadvanced ""; xl_use_area "Define FPGA area for resource estimation"; xl_area "FPGA area [slices, FFs, BRAMs, LUTs, IOBs, emb. mults, TBUFs]"; has_advanced_control ""; sggui_pos ""; block_type ""; block_version ""; sg_icon_stat ""; sg_mask_display ""; sg_list_contents ""; sg_blockgui_xml ""
      mask help: Xilinx Single Port Read-Only Memory
      mask init:
      | try
      |   tmp_gcb = gcb;
      |   tmp_gcbh = gcbh;
      |   if (strcmp('SysGenIndex',get_param(bdroot(tmp_gcbh),'tag')) && ~isempty(regexp(bdroot(tmp_gcb), '^xbs', 'once')))
      |     return;
      |   end;
      |   xlMungeMaskParams;
      |   block_config = 'sysgen_blockset:SPROM_config';
      | 
      |   block_type='sprom';
      | 
      |   serialized_declarations = '{''arith_type''=>''Int'',''bin_pt''=>''Int'',''bool''=>''Int'',''depth''=>''Int'',''distributed_mem''=>''Int'',''en''=>''Bool'',''exp_width''=>''Int'',''frac_width''=>''Int'',''gui_display_data_type''=>''Int'',''initVector''=>''DoubleVector'',''init_reg''=>''Double'',''latency''=>''Int'',''n_bits''=>''Int'',''optimize''=>''Int'',''preci_type''=>''Int'',''rst''=>''Bool'',''use_rpm''=>''Int'',''block_type''=>''String''}';
      |   ptable_ = xlblockprep(get_param(tmp_gcb, 'MaskWSVariables'));
      |   try
      |     xlBlockMoveCallback(tmp_gcbh);
      |   catch 
      |      clear global xl_updateicon_recursion_guard;
      |   end;
      | catch
      |   global dbgsysgen;
      |   if(~isempty(dbgsysgen) && dbgsysgen)
      |     e = regexprep(lasterr, '\n', '\nError: ');
      |     disp(['Error: While running MaskInit code on block ' tmp_gcb ': ' e]);
      |     error(e);
      |   end
      | end
      settings: CopyFcn=xlBlockMoveCallback(gcbh);  DeleteFcn=xlDestroyGui(gcbh);  ModelCloseFcn=xlDestroyGui(gcbh);  PreSaveFcn=xlBlockPreSaveCallback(gcbh);  PostSaveFcn=xlBlockPostSaveCallback(gcbh);  DestroyFcn=xlDestroyGui(gcbh);  OpenFcn=xlOpenGui(gcbh, 'sprom_gui.xml', @spromenablement, @spromaction)  CloseFcn=xlDestroyGui(gcbh);  MoveFcn=xlBlockMoveCallback(gcbh);
      mask Help: eval('');xlDoc('-book','sysgen','-topic','ROM');
      mask StyleString: edit,edit,edit,popup(Distributed memory|Block RAM),edit,checkbox,edit,edit,checkbox,edit,edit,popup(Boolean|Fixed-point|Floating-point),edit,popup(Boolean|Unsigned|Signed  (2's comp)|Floating-point),edit,edit,edit,popup(Single|Double|Custom),edit,edit,edit,checkbox,edit,popup(Area|Speed|Power),edit,checkbox,edit,checkbox,edit,edit,edit,edit,edit,edit,edit,edit,edit
      mask Display:
      | fprintf('','COMMENT: begin icon graphics');
      | patch([0 60 60 0 0 ],[0 0 56 56 0 ],[0.77 0.82 0.91 ]);
      | plot([0 60 60 0 0 ],[0 0 56 56 0 ]);
      | patch([12.2 23.76 31.76 39.76 47.76 31.76 20.2 12.2 ],[36.88 36.88 44.88 36.88 44.88 44.88 44.88 36.88 ],[1 1 1 ]);
      | patch([20.2 31.76 23.76 12.2 20.2 ],[28.88 28.88 36.88 36.88 28.88 ],[0.931 0.946 0.973 ]);
      | patch([12.2 23.76 31.76 20.2 12.2 ],[20.88 20.88 28.88 28.88 20.88 ],[1 1 1 ]);
      | patch([20.2 47.76 39.76 31.76 23.76 12.2 20.2 ],[12.88 12.88 20.88 12.88 20.88 20.88 12.88 ],[0.931 0.946 0.973 ]);
      | fprintf('','COMMENT: end icon graphics');
      | fprintf('','COMMENT: begin icon text');
      | color('black');port_label('input',1,'addr');
      | 
      | color('black');disp('z^{-1}','texmode','on');
      | fprintf('','COMMENT: end icon text');
  "RS Decoder v5_1 " : S-Function  LoadFcn=xlBlockLoadCallback(gcbh);  FunctionName=sysgen  Parameters=ptable_  EnableBusSupport=off  mask(Xilinx Reed-Solomon Decoder Block){infoedit=Decodes systematically encoded RS codes. The decoder supports marking received data symbols as erasures., code_spec_sgadvanced=, code_spec=DVB, num_channels=1, clocks_per_symbol=1, erase_sgadvanced=, erase=off, data_del_sgadvanced=, data_del=off, n_in_sgadvanced=, n_in=off, rst_sgadvanced=, rst=off, en_sgadvanced=, en=off, sym_width=8, nn=204, kk=188, poly_char=[ 1 0 0 0 1 1 1 0 1], gen_start=0, scale=1, mem_style_sgadvanced=, mem_style=Automatic, opt_mode_sgadvanced=, opt_mode=Speed, self_recovering_sgadvanced=, self_recovering=off, use_rpm_sgadvanced=, use_rpm=off, xl_use_area_sgadvanced=, xl_use_area=off, xl_area=[0,0,0,0,0,0,0], core_version=5.1, has_advanced_control=0, sggui_pos=-1,-1,-1,-1, block_type=rsdecode, block_version=, sg_icon_stat=85,156,-1,-1,white,green,0,07734,right,,[ ],[ ], sg_mask_display=|, sg_list_contents=, sg_blockgui_xml=}
      mask sg_mask_display=|
      | fprintf('','COMMENT: begin icon graphics');
      | patch([0 85 85 0 0 ],[0 0 156 156 0 ],[0.72 0.84 0.7 ]);
      | plot([0 85 85 0 0 ],[0 0 156 156 0 ]);
      | patch([15.3 32.64 44.64 56.64 68.64 44.64 27.3 15.3 ],[91.32 91.32 103.32 91.32 103.32 103.32 103.32 91.32 ],[1 1 1 ]);
      | patch([27.3 44.64 32.64 15.3 27.3 ],[79.32 79.32 91.32 91.32 79.32 ],[0.916 0.952 0.91 ]);
      | patch([15.3 32.64 44.64 27.3 15.3 ],[67.32 67.32 79.32 79.32 67.32 ],[1 1 1 ]);
      | patch([27.3 68.64 56.64 44.64 32.64 15.3 27.3 ],[55.32 55.32 67.32 55.32 67.32 67.32 55.32 ],[0.916 0.952 0.91 ]);
      | fprintf('','COMMENT: end icon graphics');
      | fprintf('','COMMENT: begin icon text');
      | fprintf('','COMMENT: end icon text');
      mask prompts: infoedit ""; code_spec_sgadvanced ""; code_spec "Code specification"; num_channels "Number of channels integer between 1 and 128"; clocks_per_symbol "Clocks per symbol"; erase_sgadvanced ""; erase "Provide erase port"; data_del_sgadvanced ""; data_del "Provide original delayed data port (<tt>data_del</tt>)"; n_in_sgadvanced ""; n_in "Provide variable block length port (<tt>n_in</tt>)"; rst_sgadvanced ""; rst "Provide synchronous reset port"; en_sgadvanced ""; en "Provide enable port"; sym_width "Symbol width integer between 3 and 12"; nn "Number of symbols per code block (n)"; kk "Number of information symbols per code block (k)"; poly_char "Field polynomial (example: [ 1 0 1 1] => x^3  +  x  +  1)"; gen_start "Generator start (log of first root of generator polynomial)"; scale "Scaling factor for generator polynomial"; mem_style_sgadvanced ""; mem_style "Memory Type"; opt_mode_sgadvanced ""; opt_mode "Optimization"; self_recovering_sgadvanced ""; self_recovering "Self recovering state machine"; use_rpm_sgadvanced ""; use_rpm "Use core placement information"; xl_use_area_sgadvanced ""; xl_use_area "Define FPGA area for resource estimation"; xl_area "FPGA area [slices, FFs, BRAMs, LUTs, IOBs, emb. mults, TBUFs]"; core_version ""; has_advanced_control ""; sggui_pos ""; block_type ""; block_version ""; sg_icon_stat ""; sg_mask_display ""; sg_list_contents ""; sg_blockgui_xml ""
      mask help: Decodes systematically encoded RS codes. The decoder supports marking received data symbols as erasures.
      mask init:
      | try
      |   tmp_gcb = gcb;
      |   tmp_gcbh = gcbh;
      |   if (strcmp('SysGenIndex',get_param(bdroot(tmp_gcbh),'tag')) && ~isempty(regexp(bdroot(tmp_gcb), '^xbs', 'once')))
      |     return;
      |   end;
      |   xlMungeMaskParams;
      |   block_config = 'sysgen_blockset:Removed_config';
      | 
      |   block_type='rsdecode';
      | nport = get_param(gcbh, 'ports');
      | nin = nport(1);
      | nout = nport(2);
      | 
      |   serialized_declarations = '{''alpha''=>''Int'',''clocks_per_symbol''=>''Int'',''code_spec''=>''Int'',''core_version''=>''String'',''data_del''=>''Int'',''en''=>''Int'',''erase''=>''Int'',''gen_start''=>''Int'',''kk''=>''Int'',''mem_style''=>''Int'',''n_in''=>''Int'',''nn''=>''Int'',''num_channels''=>''Int'',''opt_mode''=>''Int'',''poly''=>''String'',''rst''=>''Int'',''scale''=>''Int'',''self_recovering''=>''Int'',''sym_width''=>''Int'',''use_rpm''=>''Int'',''block_type''=>''String'',''nin''=>''Double'',''nout''=>''Double''}';
      |   xlrsdecode_init();
      |   ptable_ = xlblockprep(get_param(tmp_gcb, 'MaskWSVariables'));
      |   try
      |     xlBlockMoveCallback(tmp_gcbh);
      |   catch 
      |      clear global xl_updateicon_recursion_guard;
      |   end;
      | catch
      |   global dbgsysgen;
      |   if(~isempty(dbgsysgen) && dbgsysgen)
      |     e = regexprep(lasterr, '\n', '\nError: ');
      |     disp(['Error: While running MaskInit code on block ' tmp_gcb ': ' e]);
      |     error(e);
      |   end
      | end
      settings: CopyFcn=xlBlockMoveCallback(gcbh);  DeleteFcn=xlDestroyGui(gcbh);  ModelCloseFcn=xlDestroyGui(gcbh);  PreSaveFcn=xlBlockPreSaveCallback(gcbh);  PostSaveFcn=xlBlockPostSaveCallback(gcbh);  DestroyFcn=xlDestroyGui(gcbh);  OpenFcn=xlOpenGui(gcbh, 'rsdecode_gui.xml', @xlremovedenablement, -1)  CloseFcn=xlDestroyGui(gcbh);  MoveFcn=xlBlockMoveCallback(gcbh);
      mask Help: eval('');xlDoc('-book','sysgen','-topic','RS_Decoder_v5_1');
      mask StyleString: edit,edit,popup(Custom|ATSC|CCSDS|DVB|IESS-308 (126)|IESS-308 (194)|IESS-308 (208)|IESS-308 (219)|IESS-308 (225)|IEEE-802.16d),edit,edit,edit,checkbox,edit,checkbox,edit,checkbox,edit,checkbox,edit,checkbox,edit,edit,edit,edit,edit,edit,edit,popup(Automatic|Block RAM|Distributed memory),edit,popup(Area|Speed),edit,checkbox,edit,checkbox,edit,checkbox,edit,edit,edit,edit,edit,edit,edit,edit,edit,edit
      mask Display:
      | fprintf('','COMMENT: begin icon graphics');
      | patch([0 85 85 0 0 ],[0 0 156 156 0 ],[0.72 0.84 0.7 ]);
      | plot([0 85 85 0 0 ],[0 0 156 156 0 ]);
      | patch([15.3 32.64 44.64 56.64 68.64 44.64 27.3 15.3 ],[91.32 91.32 103.32 91.32 103.32 103.32 103.32 91.32 ],[1 1 1 ]);
      | patch([27.3 44.64 32.64 15.3 27.3 ],[79.32 79.32 91.32 91.32 79.32 ],[0.916 0.952 0.91 ]);
      | patch([15.3 32.64 44.64 27.3 15.3 ],[67.32 67.32 79.32 79.32 67.32 ],[1 1 1 ]);
      | patch([27.3 68.64 56.64 44.64 32.64 15.3 27.3 ],[55.32 55.32 67.32 55.32 67.32 67.32 55.32 ],[0.916 0.952 0.91 ]);
      | fprintf('','COMMENT: end icon graphics');
      | fprintf('','COMMENT: begin icon text');
      | fprintf('','COMMENT: end icon text');
  "RS Decoder v6_0 " : S-Function  LoadFcn=xlBlockLoadCallback(gcbh);  FunctionName=sysgen  Parameters=ptable_  EnableBusSupport=off  mask(Xilinx Reed-Solomon Decoder Block){infoedit=Decodes systematically encoded RS codes. The decoder supports marking received data symbols as erasures., code_spec_sgadvanced=, code_spec=DVB, num_channels=1, clocks_per_symbol=1, erase_sgadvanced=, erase=off, data_del_sgadvanced=, data_del=off, n_in_sgadvanced=, n_in=off, rst_sgadvanced=, rst=off, en_sgadvanced=, en=off, sym_width=8, nn=204, kk=188, poly_char=[ 1 0 0 0 1 1 1 0 1], gen_start=0, scale=1, mem_style_sgadvanced=, mem_style=Automatic, opt_mode_sgadvanced=, opt_mode=Speed, self_recovering_sgadvanced=, self_recovering=off, xl_use_area_sgadvanced=, xl_use_area=off, xl_area=[0,0,0,0,0,0,0], core_version=6.0, has_advanced_control=0, sggui_pos=-1,-1,-1,-1, block_type=rsdecode60, block_version=, sg_icon_stat=85,156,-1,-1,white,green,0,07734,right,,[ ],[ ], sg_mask_display=|, sg_list_contents=, sg_blockgui_xml=}
      mask sg_mask_display=|
      | fprintf('','COMMENT: begin icon graphics');
      | patch([0 85 85 0 0 ],[0 0 156 156 0 ],[0.72 0.84 0.7 ]);
      | plot([0 85 85 0 0 ],[0 0 156 156 0 ]);
      | patch([15.3 32.64 44.64 56.64 68.64 44.64 27.3 15.3 ],[91.32 91.32 103.32 91.32 103.32 103.32 103.32 91.32 ],[1 1 1 ]);
      | patch([27.3 44.64 32.64 15.3 27.3 ],[79.32 79.32 91.32 91.32 79.32 ],[0.916 0.952 0.91 ]);
      | patch([15.3 32.64 44.64 27.3 15.3 ],[67.32 67.32 79.32 79.32 67.32 ],[1 1 1 ]);
      | patch([27.3 68.64 56.64 44.64 32.64 15.3 27.3 ],[55.32 55.32 67.32 55.32 67.32 67.32 55.32 ],[0.916 0.952 0.91 ]);
      | fprintf('','COMMENT: end icon graphics');
      | fprintf('','COMMENT: begin icon text');
      | fprintf('','COMMENT: end icon text');
      mask prompts: infoedit ""; code_spec_sgadvanced ""; code_spec "Code specification"; num_channels "Number of channels integer between 1 and 128"; clocks_per_symbol "Clocks per symbol"; erase_sgadvanced ""; erase "Provide erase port"; data_del_sgadvanced ""; data_del "Provide original delayed data port (<tt>data_del</tt>)"; n_in_sgadvanced ""; n_in "Provide variable block length port (<tt>n_in</tt>)"; rst_sgadvanced ""; rst "Provide synchronous reset port"; en_sgadvanced ""; en "Provide enable port"; sym_width "Symbol width integer between 3 and 12"; nn "Number of symbols per code block (n)"; kk "Number of information symbols per code block (k)"; poly_char "Field polynomial (example: [ 1 0 1 1] => x^3  +  x  +  1)"; gen_start "Generator start (log of first root of generator polynomial)"; scale "Scaling factor for generator polynomial"; mem_style_sgadvanced ""; mem_style "Memory Type"; opt_mode_sgadvanced ""; opt_mode "Optimization"; self_recovering_sgadvanced ""; self_recovering "Self recovering state machine"; xl_use_area_sgadvanced ""; xl_use_area "Define FPGA area for resource estimation"; xl_area "FPGA area [slices, FFs, BRAMs, LUTs, IOBs, emb. mults, TBUFs]"; core_version ""; has_advanced_control ""; sggui_pos ""; block_type ""; block_version ""; sg_icon_stat ""; sg_mask_display ""; sg_list_contents ""; sg_blockgui_xml ""
      mask help: Decodes systematically encoded RS codes. The decoder supports marking received data symbols as erasures.
      mask init:
      | try
      |   tmp_gcb = gcb;
      |   tmp_gcbh = gcbh;
      |   if (strcmp('SysGenIndex',get_param(bdroot(tmp_gcbh),'tag')) && ~isempty(regexp(bdroot(tmp_gcb), '^xbs', 'once')))
      |     return;
      |   end;
      |   xlMungeMaskParams;
      |   block_config = 'sysgen_blockset:Removed_config';
      | 
      |   block_type='rsdecode60';
      | nport = get_param(gcbh, 'ports');
      | nin = nport(1);
      | nout = nport(2);
      | 
      |   serialized_declarations = '{''alpha''=>''Int'',''clocks_per_symbol''=>''Int'',''code_spec''=>''Int'',''core_version''=>''String'',''data_del''=>''Int'',''en''=>''Int'',''erase''=>''Int'',''gen_start''=>''Int'',''kk''=>''Int'',''mem_style''=>''Int'',''n_in''=>''Int'',''nn''=>''Int'',''num_channels''=>''Int'',''opt_mode''=>''Int'',''poly''=>''String'',''rst''=>''Int'',''scale''=>''Int'',''self_recovering''=>''Int'',''sym_width''=>''Int'',''block_type''=>''String'',''nin''=>''Double'',''nout''=>''Double''}';
      |   xlrsdecode_init();
      |   ptable_ = xlblockprep(get_param(tmp_gcb, 'MaskWSVariables'));
      |   try
      |     xlBlockMoveCallback(tmp_gcbh);
      |   catch 
      |      clear global xl_updateicon_recursion_guard;
      |   end;
      | catch
      |   global dbgsysgen;
      |   if(~isempty(dbgsysgen) && dbgsysgen)
      |     e = regexprep(lasterr, '\n', '\nError: ');
      |     disp(['Error: While running MaskInit code on block ' tmp_gcb ': ' e]);
      |     error(e);
      |   end
      | end
      settings: CopyFcn=xlBlockMoveCallback(gcbh);  DeleteFcn=xlDestroyGui(gcbh);  ModelCloseFcn=xlDestroyGui(gcbh);  PreSaveFcn=xlBlockPreSaveCallback(gcbh);  PostSaveFcn=xlBlockPostSaveCallback(gcbh);  DestroyFcn=xlDestroyGui(gcbh);  OpenFcn=xlOpenGui(gcbh, 'rsdecodev60_gui.xml', @xlremovedenablement, -1)  CloseFcn=xlDestroyGui(gcbh);  MoveFcn=xlBlockMoveCallback(gcbh);
      mask Help: eval('');xlDoc('-book','sysgen','-topic','RS_Decoder_v6_0');
      mask StyleString: edit,edit,popup(Custom|ATSC|CCSDS|DVB|IESS-308 (126)|IESS-308 (194)|IESS-308 (208)|IESS-308 (219)|IESS-308 (225)|IEEE-802.16d),edit,edit,edit,checkbox,edit,checkbox,edit,checkbox,edit,checkbox,edit,checkbox,edit,edit,edit,edit,edit,edit,edit,popup(Automatic|Block RAM|Distributed memory),edit,popup(Area|Speed),edit,checkbox,edit,checkbox,edit,edit,edit,edit,edit,edit,edit,edit,edit,edit
      mask Display:
      | fprintf('','COMMENT: begin icon graphics');
      | patch([0 85 85 0 0 ],[0 0 156 156 0 ],[0.72 0.84 0.7 ]);
      | plot([0 85 85 0 0 ],[0 0 156 156 0 ]);
      | patch([15.3 32.64 44.64 56.64 68.64 44.64 27.3 15.3 ],[91.32 91.32 103.32 91.32 103.32 103.32 103.32 91.32 ],[1 1 1 ]);
      | patch([27.3 44.64 32.64 15.3 27.3 ],[79.32 79.32 91.32 91.32 79.32 ],[0.916 0.952 0.91 ]);
      | patch([15.3 32.64 44.64 27.3 15.3 ],[67.32 67.32 79.32 79.32 67.32 ],[1 1 1 ]);
      | patch([27.3 68.64 56.64 44.64 32.64 15.3 27.3 ],[55.32 55.32 67.32 55.32 67.32 67.32 55.32 ],[0.916 0.952 0.91 ]);
      | fprintf('','COMMENT: end icon graphics');
      | fprintf('','COMMENT: begin icon text');
      | fprintf('','COMMENT: end icon text');
  "RS Encoder v5_0 " : S-Function  LoadFcn=xlBlockLoadCallback(gcbh);  FunctionName=sysgen  Parameters=ptable_  EnableBusSupport=off  mask(Xilinx Reed-Solomon Encoder Block){infoedit=Systematic Reed-Solomon (RS) encoder. The encoder transforms each block of k information symbols presented serially at the input port to a block of n symbols presented serially at the output port., code_spec_sgadvanced=, code_spec=DVB, num_channels=1, r_in_sgadvanced=, r_in=off, n_in_sgadvanced=, n_in=off, nd_sgadvanced=, nd=off, rdy_sgadvanced=, rdy=off, rfd_sgadvanced=, rfd=off, rffd_sgadvanced=, rffd=off, rst_sgadvanced=, rst=off, en_sgadvanced=, en=off, sym_width=8, nn=204, kk=188, poly_char=[1 0 0 0 1 1 1 0 1], gen_start=0, scale=1, dbl_ovrd_sgadvanced=, dbl_ovrd=off, mem_style_sgadvanced=, mem_style=Automatic, sym_generator_sgadvanced=, sym_generator=Optimized for area, use_rpm_sgadvanced=, use_rpm=off, xl_use_area_sgadvanced=, xl_use_area=off, xl_area=[0,0,0,0,0,0,0], core_version=5.0, has_advanced_control=0, sggui_pos=-1,-1,-1,-1, block_type=rsencode, block_version=, sg_icon_stat=95,142,-1,-1,white,green,0,07734,right,,[ ],[ ], sg_mask_display=|, sg_list_contents=, sg_blockgui_xml=}
      mask sg_mask_display=|
      | fprintf('','COMMENT: begin icon graphics');
      | patch([0 95 95 0 0 ],[0 0 142 142 0 ],[0.72 0.84 0.7 ]);
      | plot([0 95 95 0 0 ],[0 0 142 142 0 ]);
      | patch([18.075 36.86 49.86 62.86 75.86 49.86 31.075 18.075 ],[85.43 85.43 98.43 85.43 98.43 98.43 98.43 85.43 ],[1 1 1 ]);
      | patch([31.075 49.86 36.86 18.075 31.075 ],[72.43 72.43 85.43 85.43 72.43 ],[0.916 0.952 0.91 ]);
      | patch([18.075 36.86 49.86 31.075 18.075 ],[59.43 59.43 72.43 72.43 59.43 ],[1 1 1 ]);
      | patch([31.075 75.86 62.86 49.86 36.86 18.075 31.075 ],[46.43 46.43 59.43 46.43 59.43 59.43 46.43 ],[0.916 0.952 0.91 ]);
      | fprintf('','COMMENT: end icon graphics');
      | fprintf('','COMMENT: begin icon text');
      | fprintf('','COMMENT: end icon text');
      mask prompts: infoedit ""; code_spec_sgadvanced ""; code_spec "Code specification"; num_channels "Number of channels (integer between 1 and 128)"; r_in_sgadvanced ""; r_in "Provide variable number of check symbols port (<tt>r_in</tt>)"; n_in_sgadvanced ""; n_in "Provide variable block Length port (<tt>n_in</tt>)"; nd_sgadvanced ""; nd "Provide new data port (<tt>nd</tt>)"; rdy_sgadvanced ""; rdy "Provide ready port (<tt>rdy</tt>)"; rfd_sgadvanced ""; rfd "Provide ready for data port (<tt>rfd</tt>)"; rffd_sgadvanced ""; rffd "Provide ready for first data port (<tt>rffd</tt>)"; rst_sgadvanced ""; rst "Provide synchronous reset port"; en_sgadvanced ""; en "Provide enable port"; sym_width "Symbol width (integer between 3 and 12)"; nn "n (number of symbols per code block)"; kk "k (number of information symbols per code block)"; poly_char "Field polynomial (example: [1 0 1 1] => x^3  +  x  +  1)"; gen_start "Generator start (log of first root of generator polynomial)"; scale "Scaling factor for generator polynomial"; dbl_ovrd_sgadvanced ""; dbl_ovrd "Override with doubles"; mem_style_sgadvanced ""; mem_style "Memory style"; sym_generator_sgadvanced ""; sym_generator "Check Symbol Generator"; use_rpm_sgadvanced ""; use_rpm "Use core placement information"; xl_use_area_sgadvanced ""; xl_use_area "Define FPGA area for resource estimation"; xl_area "FPGA area [slices, FFs, BRAMs, LUTs, IOBs, emb. mults, TBUFs]"; core_version ""; has_advanced_control ""; sggui_pos ""; block_type ""; block_version ""; sg_icon_stat ""; sg_mask_display ""; sg_list_contents ""; sg_blockgui_xml ""
      mask help: Systematic Reed-Solomon (RS) encoder. The encoder transforms each block of k information symbols presented serially at the input port to a block of n symbols presented serially at the output port.
      mask init:
      | try
      |   tmp_gcb = gcb;
      |   tmp_gcbh = gcbh;
      |   if (strcmp('SysGenIndex',get_param(bdroot(tmp_gcbh),'tag')) && ~isempty(regexp(bdroot(tmp_gcb), '^xbs', 'once')))
      |     return;
      |   end;
      |   xlMungeMaskParams;
      |   block_config = 'sysgen_blockset:Removed_config';
      | 
      |   block_type='rsencode';
      | nport = get_param(gcbh, 'ports');
      | nin = nport(1);
      | nout = nport(2);
      | 
      |   serialized_declarations = '{''alpha''=>''Int'',''code_spec''=>''Int'',''core_version''=>''String'',''en''=>''Bool'',''gen_start''=>''Int'',''kk''=>''Int'',''mem_style''=>''Int'',''n_in''=>''Bool'',''nd''=>''Bool'',''nn''=>''Int'',''num_channels''=>''Int'',''poly''=>''String'',''r_in''=>''Bool'',''rdy''=>''Bool'',''rfd''=>''Bool'',''rffd''=>''Bool'',''rst''=>''Bool'',''scale''=>''Int'',''sym_generator''=>''Int'',''sym_width''=>''Int'',''use_rpm''=>''Bool'',''block_type''=>''String'',''nin''=>''Double'',''nout''=>''Double''}';
      |   xlrsencode_init();
      |   ptable_ = xlblockprep(get_param(tmp_gcb, 'MaskWSVariables'));
      |   try
      |     xlBlockMoveCallback(tmp_gcbh);
      |   catch 
      |      clear global xl_updateicon_recursion_guard;
      |   end;
      | catch
      |   global dbgsysgen;
      |   if(~isempty(dbgsysgen) && dbgsysgen)
      |     e = regexprep(lasterr, '\n', '\nError: ');
      |     disp(['Error: While running MaskInit code on block ' tmp_gcb ': ' e]);
      |     error(e);
      |   end
      | end
      settings: CopyFcn=xlBlockMoveCallback(gcbh);  DeleteFcn=xlDestroyGui(gcbh);  ModelCloseFcn=xlDestroyGui(gcbh);  PreSaveFcn=xlBlockPreSaveCallback(gcbh);  PostSaveFcn=xlBlockPostSaveCallback(gcbh);  DestroyFcn=xlDestroyGui(gcbh);  OpenFcn=xlOpenGui(gcbh, 'rsencode_gui.xml', @xlremovedenablement, -1)  CloseFcn=xlDestroyGui(gcbh);  MoveFcn=xlBlockMoveCallback(gcbh);
      mask Help: eval('');xlDoc('-book','sysgen','-topic','RS_Encoder_v5_0');
      mask StyleString: edit,edit,popup(Custom|ATSC|CCSDS|DVB|IESS-308 (126)|IESS-308 (194)|IESS-308 (208)|IESS-308 (219)|IESS-308 (225)|ITU J.83 Annex B),edit,edit,checkbox,edit,checkbox,edit,checkbox,edit,checkbox,edit,checkbox,edit,checkbox,edit,checkbox,edit,checkbox,edit,edit,edit,edit,edit,edit,edit,checkbox,edit,popup(Automatic|Block|Distributed),edit,popup(Optimized for area|Optimized for flexibility),edit,checkbox,edit,checkbox,edit,edit,edit,edit,edit,edit,edit,edit,edit,edit
      mask Display:
      | fprintf('','COMMENT: begin icon graphics');
      | patch([0 95 95 0 0 ],[0 0 142 142 0 ],[0.72 0.84 0.7 ]);
      | plot([0 95 95 0 0 ],[0 0 142 142 0 ]);
      | patch([18.075 36.86 49.86 62.86 75.86 49.86 31.075 18.075 ],[85.43 85.43 98.43 85.43 98.43 98.43 98.43 85.43 ],[1 1 1 ]);
      | patch([31.075 49.86 36.86 18.075 31.075 ],[72.43 72.43 85.43 85.43 72.43 ],[0.916 0.952 0.91 ]);
      | patch([18.075 36.86 49.86 31.075 18.075 ],[59.43 59.43 72.43 72.43 59.43 ],[1 1 1 ]);
      | patch([31.075 75.86 62.86 49.86 36.86 18.075 31.075 ],[46.43 46.43 59.43 46.43 59.43 59.43 46.43 ],[0.916 0.952 0.91 ]);
      | fprintf('','COMMENT: end icon graphics');
      | fprintf('','COMMENT: begin icon text');
      | fprintf('','COMMENT: end icon text');
  "RS Encoder v6_0 " : S-Function  LoadFcn=xlBlockLoadCallback(gcbh);  FunctionName=sysgen  Parameters=ptable_  EnableBusSupport=off  mask(Xilinx Reed-Solomon Encoder Block){infoedit=Systematic Reed-Solomon (RS) encoder. The encoder transforms each block of k information symbols presented serially at the input port to a block of n symbols presented serially at the output port., code_spec_sgadvanced=, code_spec=DVB, num_channels=1, r_in_sgadvanced=, r_in=off, n_in_sgadvanced=, n_in=off, nd_sgadvanced=, nd=off, rdy_sgadvanced=, rdy=off, rfd_sgadvanced=, rfd=off, rffd_sgadvanced=, rffd=off, rst_sgadvanced=, rst=off, en_sgadvanced=, en=off, sym_width=8, nn=204, kk=188, poly_char=[1 0 0 0 1 1 1 0 1], gen_start=0, scale=1, dbl_ovrd_sgadvanced=, dbl_ovrd=off, mem_style_sgadvanced=, mem_style=Automatic, sym_generator_sgadvanced=, sym_generator=Optimized for area, use_rpm_sgadvanced=, use_rpm=off, xl_use_area_sgadvanced=, xl_use_area=off, xl_area=[0,0,0,0,0,0,0], core_version=6.0, has_advanced_control=0, sggui_pos=-1,-1,-1,-1, block_type=rsencodev60, block_version=, sg_icon_stat=95,142,-1,-1,white,green,0,07734,right,,[ ],[ ], sg_mask_display=|, sg_list_contents=, sg_blockgui_xml=}
      mask sg_mask_display=|
      | fprintf('','COMMENT: begin icon graphics');
      | patch([0 95 95 0 0 ],[0 0 142 142 0 ],[0.72 0.84 0.7 ]);
      | plot([0 95 95 0 0 ],[0 0 142 142 0 ]);
      | patch([18.075 36.86 49.86 62.86 75.86 49.86 31.075 18.075 ],[85.43 85.43 98.43 85.43 98.43 98.43 98.43 85.43 ],[1 1 1 ]);
      | patch([31.075 49.86 36.86 18.075 31.075 ],[72.43 72.43 85.43 85.43 72.43 ],[0.916 0.952 0.91 ]);
      | patch([18.075 36.86 49.86 31.075 18.075 ],[59.43 59.43 72.43 72.43 59.43 ],[1 1 1 ]);
      | patch([31.075 75.86 62.86 49.86 36.86 18.075 31.075 ],[46.43 46.43 59.43 46.43 59.43 59.43 46.43 ],[0.916 0.952 0.91 ]);
      | fprintf('','COMMENT: end icon graphics');
      | fprintf('','COMMENT: begin icon text');
      | fprintf('','COMMENT: end icon text');
      mask prompts: infoedit ""; code_spec_sgadvanced ""; code_spec "Code specification"; num_channels "Number of channels (integer between 1 and 128)"; r_in_sgadvanced ""; r_in "Provide variable number of check symbols port (<tt>r_in</tt>)"; n_in_sgadvanced ""; n_in "Provide variable block Length port (<tt>n_in</tt>)"; nd_sgadvanced ""; nd "Provide new data port (<tt>nd</tt>)"; rdy_sgadvanced ""; rdy "Provide ready port (<tt>rdy</tt>)"; rfd_sgadvanced ""; rfd "Provide ready for data port (<tt>rfd</tt>)"; rffd_sgadvanced ""; rffd "Provide ready for first data port (<tt>rffd</tt>)"; rst_sgadvanced ""; rst "Provide synchronous reset port"; en_sgadvanced ""; en "Provide enable port"; sym_width "Symbol width (integer between 3 and 12)"; nn "n (number of symbols per code block)"; kk "k (number of information symbols per code block)"; poly_char "Field polynomial (example: [1 0 1 1] => x^3  +  x  +  1)"; gen_start "Generator start (log of first root of generator polynomial)"; scale "Scaling factor for generator polynomial"; dbl_ovrd_sgadvanced ""; dbl_ovrd "Override with doubles"; mem_style_sgadvanced ""; mem_style "Memory style"; sym_generator_sgadvanced ""; sym_generator "Check Symbol Generator"; use_rpm_sgadvanced ""; use_rpm "Use core placement information"; xl_use_area_sgadvanced ""; xl_use_area "Define FPGA area for resource estimation"; xl_area "FPGA area [slices, FFs, BRAMs, LUTs, IOBs, emb. mults, TBUFs]"; core_version ""; has_advanced_control ""; sggui_pos ""; block_type ""; block_version ""; sg_icon_stat ""; sg_mask_display ""; sg_list_contents ""; sg_blockgui_xml ""
      mask help: Systematic Reed-Solomon (RS) encoder. The encoder transforms each block of k information symbols presented serially at the input port to a block of n symbols presented serially at the output port.
      mask init:
      | try
      |   tmp_gcb = gcb;
      |   tmp_gcbh = gcbh;
      |   if (strcmp('SysGenIndex',get_param(bdroot(tmp_gcbh),'tag')) && ~isempty(regexp(bdroot(tmp_gcb), '^xbs', 'once')))
      |     return;
      |   end;
      |   xlMungeMaskParams;
      |   block_config = 'sysgen_blockset:Removed_config';
      | 
      |   block_type='rsencodev60';
      | nport = get_param(gcbh, 'ports');
      | nin = nport(1);
      | nout = nport(2);
      | 
      |   serialized_declarations = '{''alpha''=>''Int'',''code_spec''=>''Int'',''core_version''=>''String'',''en''=>''Bool'',''gen_start''=>''Int'',''kk''=>''Int'',''mem_style''=>''Int'',''n_in''=>''Bool'',''nd''=>''Bool'',''nn''=>''Int'',''num_channels''=>''Int'',''poly''=>''String'',''r_in''=>''Bool'',''rdy''=>''Bool'',''rfd''=>''Bool'',''rffd''=>''Bool'',''rst''=>''Bool'',''scale''=>''Int'',''sym_generator''=>''Int'',''sym_width''=>''Int'',''use_rpm''=>''Bool'',''block_type''=>''String'',''nin''=>''Double'',''nout''=>''Double''}';
      |   xlrsencode_init();
      |   ptable_ = xlblockprep(get_param(tmp_gcb, 'MaskWSVariables'));
      |   try
      |     xlBlockMoveCallback(tmp_gcbh);
      |   catch 
      |      clear global xl_updateicon_recursion_guard;
      |   end;
      | catch
      |   global dbgsysgen;
      |   if(~isempty(dbgsysgen) && dbgsysgen)
      |     e = regexprep(lasterr, '\n', '\nError: ');
      |     disp(['Error: While running MaskInit code on block ' tmp_gcb ': ' e]);
      |     error(e);
      |   end
      | end
      settings: CopyFcn=xlBlockMoveCallback(gcbh);  DeleteFcn=xlDestroyGui(gcbh);  ModelCloseFcn=xlDestroyGui(gcbh);  PreSaveFcn=xlBlockPreSaveCallback(gcbh);  PostSaveFcn=xlBlockPostSaveCallback(gcbh);  DestroyFcn=xlDestroyGui(gcbh);  OpenFcn=xlOpenGui(gcbh, 'rsencodev60_gui.xml', @xlremovedenablement, -1)  CloseFcn=xlDestroyGui(gcbh);  MoveFcn=xlBlockMoveCallback(gcbh);
      mask Help: eval('');xlDoc('-book','sysgen','-topic','RS_Encoder_v6_0');
      mask StyleString: edit,edit,popup(Custom|ATSC|CCSDS|DVB|IESS-308 (126)|IESS-308 (194)|IESS-308 (208)|IESS-308 (219)|IESS-308 (225)|ITU J.83 Annex B),edit,edit,checkbox,edit,checkbox,edit,checkbox,edit,checkbox,edit,checkbox,edit,checkbox,edit,checkbox,edit,checkbox,edit,edit,edit,edit,edit,edit,edit,checkbox,edit,popup(Automatic|Block|Distributed),edit,popup(Optimized for area|Optimized for flexibility),edit,checkbox,edit,checkbox,edit,edit,edit,edit,edit,edit,edit,edit,edit,edit
      mask Display:
      | fprintf('','COMMENT: begin icon graphics');
      | patch([0 95 95 0 0 ],[0 0 142 142 0 ],[0.72 0.84 0.7 ]);
      | plot([0 95 95 0 0 ],[0 0 142 142 0 ]);
      | patch([18.075 36.86 49.86 62.86 75.86 49.86 31.075 18.075 ],[85.43 85.43 98.43 85.43 98.43 98.43 98.43 85.43 ],[1 1 1 ]);
      | patch([31.075 49.86 36.86 18.075 31.075 ],[72.43 72.43 85.43 85.43 72.43 ],[0.916 0.952 0.91 ]);
      | patch([18.075 36.86 49.86 31.075 18.075 ],[59.43 59.43 72.43 72.43 59.43 ],[1 1 1 ]);
      | patch([31.075 75.86 62.86 49.86 36.86 18.075 31.075 ],[46.43 46.43 59.43 46.43 59.43 59.43 46.43 ],[0.916 0.952 0.91 ]);
      | fprintf('','COMMENT: end icon graphics');
      | fprintf('','COMMENT: begin icon text');
      | fprintf('','COMMENT: end icon text');
  Reciprocal : S-Function  LoadFcn=xlBlockLoadCallback(gcbh);  FunctionName=sysgen  Parameters=ptable_  EnableBusSupport=off  mask(Xilinx Reciprocal Block){infoedit=Blocking: Wait for data on all inputs, allow back-pressure.<br>NonBlocking: operate every cycle in which all inputs are valid, no back-pressure., flow_control=NonBlocking, axi_optimize_goal=Resources, latency=0, has_a_tlast=off, has_a_tuser=off, en=off, has_result_tready=off, has_underflow=off, has_divide_by_zero=off, xl_use_area_sgadvanced=, xl_use_area=off, xl_area=[0,0,0,0,0,0,0], fpo_op_type=reciprocal, rate=1, has_b_tlast=false, has_b_tuser=false, result_tlast_behv=1, has_overflow=false, has_invalid_op=false, has_advanced_control=0, sggui_pos=-1,-1,-1,-1, block_type=reciprocal, block_version=, sg_icon_stat=55,54,1,1,white,blue,0,6ed2cfaf,right,,[ ],[ ], sg_mask_display=|, sg_list_contents=, sg_blockgui_xml=}
      mask sg_mask_display=|
      | fprintf('','COMMENT: begin icon graphics');
      | patch([0 55 55 0 0 ],[0 0 54 54 0 ],[0.77 0.82 0.91 ]);
      | plot([0 55 55 0 0 ],[0 0 54 54 0 ]);
      | patch([11.425 21.54 28.54 35.54 42.54 28.54 18.425 11.425 ],[34.77 34.77 41.77 34.77 41.77 41.77 41.77 34.77 ],[1 1 1 ]);
      | patch([18.425 28.54 21.54 11.425 18.425 ],[27.77 27.77 34.77 34.77 27.77 ],[0.931 0.946 0.973 ]);
      | patch([11.425 21.54 28.54 18.425 11.425 ],[20.77 20.77 27.77 27.77 20.77 ],[1 1 1 ]);
      | patch([18.425 42.54 35.54 28.54 21.54 11.425 18.425 ],[13.77 13.77 20.77 13.77 20.77 20.77 13.77 ],[0.931 0.946 0.973 ]);
      | fprintf('','COMMENT: end icon graphics');
      | fprintf('','COMMENT: begin icon text');
      | color('black');port_label('input',1,'a');
      | color('black');port_label('output',1,'op');
      | fprintf('','COMMENT: end icon text');
      mask prompts: infoedit ""; flow_control "Flow Control"; axi_optimize_goal "Optimize Goal"; has_a_tlast "Has TLAST"; has_a_tuser "Has TUSER"; en "Provide enable port"; has_result_tready "Has Result TREADY"; has_underflow "UNDERFLOW"; has_divide_by_zero "DIVIDE_BY_ZERO"; xl_use_area_sgadvanced ""; xl_use_area "Define FPGA area for resource estimation"; xl_area "FPGA area [slices, FFs, BRAMs, LUTs, IOBs, emb. mults, TBUFs]"; fpo_op_type ""; rate ""; has_b_tlast ""; has_b_tuser ""; result_tlast_behv ""; has_overflow ""; has_invalid_op ""; has_advanced_control ""; sggui_pos ""; block_type ""; block_version ""; sg_icon_stat ""; sg_mask_display ""; sg_list_contents ""; sg_blockgui_xml ""
      mask help:
      | Blocking: Wait for data on all inputs, allow back-pressure.
      | NonBlocking: operate every cycle in which all inputs are valid, no back-pressure.
      mask init:
      | try
      |   tmp_gcb = gcb;
      |   tmp_gcbh = gcbh;
      |   if (strcmp('SysGenIndex',get_param(bdroot(tmp_gcbh),'tag')) && ~isempty(regexp(bdroot(tmp_gcb), '^xbs', 'once')))
      |     return;
      |   end;
      |   xlMungeMaskParams;
      |   block_config = 'sysgen:FPOBlockDescriptor_config';
      | 
      |   block_type='reciprocal';
      | 
      |   serialized_declarations = '{''axi_optimize_goal''=>''String'',''en''=>''Bool'',''flow_control''=>''String'',''fpo_op_type''=>''String'',''has_a_tlast''=>''Bool'',''has_a_tuser''=>''Bool'',''has_b_tlast''=>''Bool'',''has_b_tuser''=>''Bool'',''has_divide_by_zero''=>''Bool'',''has_invalid_op''=>''Bool'',''has_overflow''=>''Bool'',''has_result_tready''=>''Bool'',''has_underflow''=>''Bool'',''latency''=>''Int'',''rate''=>''Int'',''result_tlast_behv''=>''Int'',''block_type''=>''String''}';
      |   ptable_ = xlblockprep(get_param(tmp_gcb, 'MaskWSVariables'));
      |   try
      |     xlBlockMoveCallback(tmp_gcbh);
      |   catch 
      |      clear global xl_updateicon_recursion_guard;
      |   end;
      | catch
      |   global dbgsysgen;
      |   if(~isempty(dbgsysgen) && dbgsysgen)
      |     e = regexprep(lasterr, '\n', '\nError: ');
      |     disp(['Error: While running MaskInit code on block ' tmp_gcb ': ' e]);
      |     error(e);
      |   end
      | end
      settings: CopyFcn=xlBlockMoveCallback(gcbh);  DeleteFcn=xlDestroyGui(gcbh);  ModelCloseFcn=xlDestroyGui(gcbh);  PreSaveFcn=xlBlockPreSaveCallback(gcbh);  PostSaveFcn=xlBlockPostSaveCallback(gcbh);  DestroyFcn=xlDestroyGui(gcbh);  OpenFcn=xlOpenGui(gcbh, 'reciprocal_gui.xml', @recenablement, @recaction)  CloseFcn=xlDestroyGui(gcbh);  MoveFcn=xlBlockMoveCallback(gcbh);
      mask Help: eval('');xlDoc('-book','sysgen','-topic','Reciprocal');
      mask StyleString: edit,popup(Blocking|NonBlocking),popup(Resources|Performance),edit,checkbox,checkbox,checkbox,checkbox,checkbox,checkbox,edit,checkbox,edit,edit,edit,edit,edit,edit,edit,edit,edit,edit,edit,edit,edit,edit,edit,edit
      mask Display:
      | fprintf('','COMMENT: begin icon graphics');
      | patch([0 55 55 0 0 ],[0 0 54 54 0 ],[0.77 0.82 0.91 ]);
      | plot([0 55 55 0 0 ],[0 0 54 54 0 ]);
      | patch([11.425 21.54 28.54 35.54 42.54 28.54 18.425 11.425 ],[34.77 34.77 41.77 34.77 41.77 41.77 41.77 34.77 ],[1 1 1 ]);
      | patch([18.425 28.54 21.54 11.425 18.425 ],[27.77 27.77 34.77 34.77 27.77 ],[0.931 0.946 0.973 ]);
      | patch([11.425 21.54 28.54 18.425 11.425 ],[20.77 20.77 27.77 27.77 20.77 ],[1 1 1 ]);
      | patch([18.425 42.54 35.54 28.54 21.54 11.425 18.425 ],[13.77 13.77 20.77 13.77 20.77 20.77 13.77 ],[0.931 0.946 0.973 ]);
      | fprintf('','COMMENT: end icon graphics');
      | fprintf('','COMMENT: begin icon text');
      | color('black');port_label('input',1,'a');
      | color('black');port_label('output',1,'op');
      | fprintf('','COMMENT: end icon text');
  Reciprocal SquareRoot : S-Function  LoadFcn=xlBlockLoadCallback(gcbh);  FunctionName=sysgen  Parameters=ptable_  EnableBusSupport=off  mask(Xilinx Reciprocal Square Root Block){infoedit=Blocking: Wait for data on all inputs, allow back-pressure.<br>NonBlocking: operate every cycle in which all inputs are valid, no back-pressure., flow_control=NonBlocking, axi_optimize_goal=Resources, latency=0, has_a_tlast=off, has_a_tuser=off, en=off, has_result_tready=off, has_invalid_op=off, has_divide_by_zero=off, xl_use_area_sgadvanced=, xl_use_area=off, xl_area=[0,0,0,0,0,0,0], fpo_op_type=rec_square_root, rate=1, has_b_tlast=false, has_b_tuser=false, result_tlast_behv=1, has_underflow=false, has_overflow=false, has_advanced_control=0, sggui_pos=-1,-1,-1,-1, block_type=recsqroot, block_version=, sg_icon_stat=55,54,1,1,white,blue,0,6ed2cfaf,right,,[ ],[ ], sg_mask_display=|, sg_list_contents=, sg_blockgui_xml=}
      mask sg_mask_display=|
      | fprintf('','COMMENT: begin icon graphics');
      | patch([0 55 55 0 0 ],[0 0 54 54 0 ],[0.77 0.82 0.91 ]);
      | plot([0 55 55 0 0 ],[0 0 54 54 0 ]);
      | patch([11.425 21.54 28.54 35.54 42.54 28.54 18.425 11.425 ],[34.77 34.77 41.77 34.77 41.77 41.77 41.77 34.77 ],[1 1 1 ]);
      | patch([18.425 28.54 21.54 11.425 18.425 ],[27.77 27.77 34.77 34.77 27.77 ],[0.931 0.946 0.973 ]);
      | patch([11.425 21.54 28.54 18.425 11.425 ],[20.77 20.77 27.77 27.77 20.77 ],[1 1 1 ]);
      | patch([18.425 42.54 35.54 28.54 21.54 11.425 18.425 ],[13.77 13.77 20.77 13.77 20.77 20.77 13.77 ],[0.931 0.946 0.973 ]);
      | fprintf('','COMMENT: end icon graphics');
      | fprintf('','COMMENT: begin icon text');
      | color('black');port_label('input',1,'a');
      | color('black');port_label('output',1,'op');
      | fprintf('','COMMENT: end icon text');
      mask prompts: infoedit ""; flow_control "Flow Control"; axi_optimize_goal "Optimize Goal"; has_a_tlast "Has TLAST"; has_a_tuser "Has TUSER"; en "Provide enable port"; has_result_tready "Has Result TREADY"; has_invalid_op "INVALID_OP"; has_divide_by_zero "DIVIDE_BY_ZERO"; xl_use_area_sgadvanced ""; xl_use_area "Define FPGA area for resource estimation"; xl_area "FPGA area [slices, FFs, BRAMs, LUTs, IOBs, emb. mults, TBUFs]"; fpo_op_type ""; rate ""; has_b_tlast ""; has_b_tuser ""; result_tlast_behv ""; has_underflow ""; has_overflow ""; has_advanced_control ""; sggui_pos ""; block_type ""; block_version ""; sg_icon_stat ""; sg_mask_display ""; sg_list_contents ""; sg_blockgui_xml ""
      mask help:
      | Blocking: Wait for data on all inputs, allow back-pressure.
      | NonBlocking: operate every cycle in which all inputs are valid, no back-pressure.
      mask init:
      | try
      |   tmp_gcb = gcb;
      |   tmp_gcbh = gcbh;
      |   if (strcmp('SysGenIndex',get_param(bdroot(tmp_gcbh),'tag')) && ~isempty(regexp(bdroot(tmp_gcb), '^xbs', 'once')))
      |     return;
      |   end;
      |   xlMungeMaskParams;
      |   block_config = 'sysgen:FPOBlockDescriptor_config';
      | 
      |   block_type='recsqroot';
      | 
      |   serialized_declarations = '{''axi_optimize_goal''=>''String'',''en''=>''Bool'',''flow_control''=>''String'',''fpo_op_type''=>''String'',''has_a_tlast''=>''Bool'',''has_a_tuser''=>''Bool'',''has_b_tlast''=>''Bool'',''has_b_tuser''=>''Bool'',''has_divide_by_zero''=>''Bool'',''has_invalid_op''=>''Bool'',''has_overflow''=>''Bool'',''has_result_tready''=>''Bool'',''has_underflow''=>''Bool'',''latency''=>''Int'',''rate''=>''Int'',''result_tlast_behv''=>''Int'',''block_type''=>''String''}';
      |   ptable_ = xlblockprep(get_param(tmp_gcb, 'MaskWSVariables'));
      |   try
      |     xlBlockMoveCallback(tmp_gcbh);
      |   catch 
      |      clear global xl_updateicon_recursion_guard;
      |   end;
      | catch
      |   global dbgsysgen;
      |   if(~isempty(dbgsysgen) && dbgsysgen)
      |     e = regexprep(lasterr, '\n', '\nError: ');
      |     disp(['Error: While running MaskInit code on block ' tmp_gcb ': ' e]);
      |     error(e);
      |   end
      | end
      settings: CopyFcn=xlBlockMoveCallback(gcbh);  DeleteFcn=xlDestroyGui(gcbh);  ModelCloseFcn=xlDestroyGui(gcbh);  PreSaveFcn=xlBlockPreSaveCallback(gcbh);  PostSaveFcn=xlBlockPostSaveCallback(gcbh);  DestroyFcn=xlDestroyGui(gcbh);  OpenFcn=xlOpenGui(gcbh, 'recsqroot_gui.xml', @recsqrootenablement, @recsqrootaction)  CloseFcn=xlDestroyGui(gcbh);  MoveFcn=xlBlockMoveCallback(gcbh);
      mask Help: eval('');xlDoc('-book','sysgen','-topic','Reciprocal_SquareRoot');
      mask StyleString: edit,popup(Blocking|NonBlocking),popup(Resources|Performance),edit,checkbox,checkbox,checkbox,checkbox,checkbox,checkbox,edit,checkbox,edit,edit,edit,edit,edit,edit,edit,edit,edit,edit,edit,edit,edit,edit,edit,edit
      mask Display:
      | fprintf('','COMMENT: begin icon graphics');
      | patch([0 55 55 0 0 ],[0 0 54 54 0 ],[0.77 0.82 0.91 ]);
      | plot([0 55 55 0 0 ],[0 0 54 54 0 ]);
      | patch([11.425 21.54 28.54 35.54 42.54 28.54 18.425 11.425 ],[34.77 34.77 41.77 34.77 41.77 41.77 41.77 34.77 ],[1 1 1 ]);
      | patch([18.425 28.54 21.54 11.425 18.425 ],[27.77 27.77 34.77 34.77 27.77 ],[0.931 0.946 0.973 ]);
      | patch([11.425 21.54 28.54 18.425 11.425 ],[20.77 20.77 27.77 27.77 20.77 ],[1 1 1 ]);
      | patch([18.425 42.54 35.54 28.54 21.54 11.425 18.425 ],[13.77 13.77 20.77 13.77 20.77 20.77 13.77 ],[0.931 0.946 0.973 ]);
      | fprintf('','COMMENT: end icon graphics');
      | fprintf('','COMMENT: begin icon text');
      | color('black');port_label('input',1,'a');
      | color('black');port_label('output',1,'op');
      | fprintf('','COMMENT: end icon text');
  "Reed-Solomon Decoder 6.1 " : S-Function  LoadFcn=xlBlockLoadCallback(gcbh);  FunctionName=sysgen  Parameters=ptable_  EnableBusSupport=off  mask(Xilinx Reed-Solomon Decoder 6.1 Block){infoedit=Reed-Solomon Decoder 6.1. Decodes systematically encoded RS codes. The decoder supports making received data symbols as erasure., code_specification_sgadvanced=, code_specification=Custom, number_of_channels=1, clocks_per_symbol=1, erase_sgadvanced=, erase=off, original_delayed_data_sgadvanced=, original_delayed_data=off, variable_block_length_sgadvanced=, variable_block_length=off, rst_sgadvanced=, rst=off, en_sgadvanced=, en=off, symbol_width_sgadvanced=, symbol_width=8, symbols_per_block=255, data_symbols=239, field_polynomial=0, generator_start=0, scaling_factor=1, memory_style_sgadvanced=, memory_style=Automatic, optimization_sgadvanced=, optimization=Area, self_recovering_sgadvanced=, self_recovering=off, xl_use_area_sgadvanced=, xl_use_area=off, xl_area=[0,0,0,0,0,0,0], ip_name=Reed-Solomon Decoder, ip_version=6.1, has_advanced_control=0, sggui_pos=-1,-1,-1,-1, block_type=rs_decoder_v6_1, block_version=, sg_icon_stat=95,142,-1,-1,white,green,0,07734,right,,[ ],[ ], sg_mask_display=|, sg_list_contents=, sg_blockgui_xml=}
      mask sg_mask_display=|
      | fprintf('','COMMENT: begin icon graphics');
      | patch([0 95 95 0 0 ],[0 0 142 142 0 ],[0.72 0.84 0.7 ]);
      | plot([0 95 95 0 0 ],[0 0 142 142 0 ]);
      | patch([18.075 36.86 49.86 62.86 75.86 49.86 31.075 18.075 ],[85.43 85.43 98.43 85.43 98.43 98.43 98.43 85.43 ],[1 1 1 ]);
      | patch([31.075 49.86 36.86 18.075 31.075 ],[72.43 72.43 85.43 85.43 72.43 ],[0.916 0.952 0.91 ]);
      | patch([18.075 36.86 49.86 31.075 18.075 ],[59.43 59.43 72.43 72.43 59.43 ],[1 1 1 ]);
      | patch([31.075 75.86 62.86 49.86 36.86 18.075 31.075 ],[46.43 46.43 59.43 46.43 59.43 59.43 46.43 ],[0.916 0.952 0.91 ]);
      | fprintf('','COMMENT: end icon graphics');
      | fprintf('','COMMENT: begin icon text');
      | fprintf('','COMMENT: end icon text');
      mask prompts: infoedit ""; code_specification_sgadvanced ""; code_specification "Code specification (Predefined settings for popular standards)"; number_of_channels "Number of channels (Symbols for each channel are interlaced on DATA_IN and DATA_OUT)"; clocks_per_symbol "Clocks per symbol (Number of clock periods per input sample. Use to reduce Processing Delay (measured in SAMPLE periods))"; erase_sgadvanced ""; original_delayed_data_sgadvanced ""; original_delayed_data "Original delayed data (DATA_DEL outputs DATA_IN with no error correction. Latency is identical to DATA_OUT)"; variable_block_length_sgadvanced ""; variable_block_length "Variable block length (Adds N_IN port)"; rst_sgadvanced ""; en_sgadvanced ""; symbol_width_sgadvanced ""; symbol_width "Symbol width (Bus width of DATA_IN and DATA_OUT)"; symbols_per_block "Symbols per block (Total number of symbols in an encoded block, including check symbols)"; data_symbols "Data symbols (Number of original information symbols in block, prior to encoding)"; field_polynomial "Field polynomial (Galois Field primitive polynomial (enter in decimal))"; generator_start "Generator start (Galois Field logarithm of the first root of the Generator Polynomial)"; scaling_factor "Scaling factor (Scaling factor for Generator Polynomial root index)"; memory_style_sgadvanced ""; memory_style "Memory style (Force core to use this style of internal memory. 'Automatic' means let core decide)"; optimization_sgadvanced ""; optimization "Optimization (Core is only slightly larger with speed setting)"; self_recovering_sgadvanced ""; self_recovering "Self recovering ('Self Recovering' adds internal sync reset if lock up detected)"; xl_use_area_sgadvanced ""; xl_use_area "Define FPGA area for resource estimation"; xl_area "FPGA area [slices, FFs, BRAMs, LUTs, IOBs, emb. mults, TBUFs]"; ip_name ""; ip_version ""; has_advanced_control ""; sggui_pos ""; block_type ""; block_version ""; sg_icon_stat ""; sg_mask_display ""; sg_list_contents ""; sg_blockgui_xml ""
      mask help: Reed-Solomon Decoder 6.1. Decodes systematically encoded RS codes. The decoder supports making received data symbols as erasure.
      mask init:
      | try
      |   tmp_gcb = gcb;
      |   tmp_gcbh = gcbh;
      |   if (strcmp('SysGenIndex',get_param(bdroot(tmp_gcbh),'tag')) && ~isempty(regexp(bdroot(tmp_gcb), '^xbs', 'once')))
      |     return;
      |   end;
      |   xlMungeMaskParams;
      |   block_config = 'sysgen_blockset:Removed_config';
      | 
      |   block_type='rs_decoder_v6_1';
      | nport = get_param(gcbh, 'ports');
      | nin = nport(1);
      | nout = nport(2);
      | 
      |   serialized_declarations = '{''clocks_per_symbol''=>''Int'',''code_specification''=>''String'',''data_symbols''=>''Int'',''en''=>''Bool'',''erase''=>''Bool'',''field_polynomial''=>''Int'',''generator_start''=>''Int'',''ip_name''=>''String'',''ip_version''=>''String'',''memory_style''=>''String'',''number_of_channels''=>''Int'',''optimization''=>''String'',''original_delayed_data''=>''Bool'',''rst''=>''Bool'',''scaling_factor''=>''Int'',''self_recovering''=>''Bool'',''symbol_width''=>''String'',''symbols_per_block''=>''Int'',''variable_block_length''=>''Bool'',''xl_use_area''=>''Bool'',''block_type''=>''String'',''nin''=>''Double'',''nout''=>''Double''}';
      |   ptable_ = xlblockprep(get_param(tmp_gcb, 'MaskWSVariables'));
      |   try
      |     xlBlockMoveCallback(tmp_gcbh);
      |   catch 
      |      clear global xl_updateicon_recursion_guard;
      |   end;
      | catch
      |   global dbgsysgen;
      |   if(~isempty(dbgsysgen) && dbgsysgen)
      |     e = regexprep(lasterr, '\n', '\nError: ');
      |     disp(['Error: While running MaskInit code on block ' tmp_gcb ': ' e]);
      |     error(e);
      |   end
      | end
      settings: CopyFcn=xlBlockMoveCallback(gcbh);  DeleteFcn=xlDestroyGui(gcbh);  ModelCloseFcn=xlDestroyGui(gcbh);  PreSaveFcn=xlBlockPreSaveCallback(gcbh);  PostSaveFcn=xlBlockPostSaveCallback(gcbh);  DestroyFcn=xlDestroyGui(gcbh);  OpenFcn=xlOpenGui(gcbh, 'rs_decoder_v6_1_gui.xml', @xlremovedenablement, -1)  CloseFcn=xlDestroyGui(gcbh);  MoveFcn=xlBlockMoveCallback(gcbh);
      mask Help: eval('');xlDoc('-book','sysgen','-topic','Reed_Solomon_Decoder_6_1');
      mask StyleString: edit,edit,popup(Custom|DVB|ATSC|CCSDS|IESS-308(All)|IESS-308(126)|IESS-308(194)|IESS-308(208)|IESS-308(219)|IESS-308(225)|IEEE-802.16),edit,edit,edit,checkbox,edit,checkbox,edit,checkbox,edit,checkbox,edit,checkbox,edit,popup(3|4|5|6|7|8|9|10|11|12),edit,edit,edit,edit,edit,edit,popup(Automatic|Block|Distributed),edit,popup(Area|Speed),edit,checkbox,edit,checkbox,edit,edit,edit,edit,edit,edit,edit,edit,edit,edit,edit
      mask Display:
      | fprintf('','COMMENT: begin icon graphics');
      | patch([0 95 95 0 0 ],[0 0 142 142 0 ],[0.72 0.84 0.7 ]);
      | plot([0 95 95 0 0 ],[0 0 142 142 0 ]);
      | patch([18.075 36.86 49.86 62.86 75.86 49.86 31.075 18.075 ],[85.43 85.43 98.43 85.43 98.43 98.43 98.43 85.43 ],[1 1 1 ]);
      | patch([31.075 49.86 36.86 18.075 31.075 ],[72.43 72.43 85.43 85.43 72.43 ],[0.916 0.952 0.91 ]);
      | patch([18.075 36.86 49.86 31.075 18.075 ],[59.43 59.43 72.43 72.43 59.43 ],[1 1 1 ]);
      | patch([31.075 75.86 62.86 49.86 36.86 18.075 31.075 ],[46.43 46.43 59.43 46.43 59.43 59.43 46.43 ],[0.916 0.952 0.91 ]);
      | fprintf('','COMMENT: end icon graphics');
      | fprintf('','COMMENT: begin icon text');
      | fprintf('','COMMENT: end icon text');
  "Reed-Solomon Decoder 7.0 " : S-Function  LoadFcn=xlBlockLoadCallback(gcbh);  FunctionName=sysgen  Parameters=ptable_  EnableBusSupport=off  mask(Xilinx Reed-Solomon Decoder 7.0  Block){code_specification=Custom, symbol_width=8, field_polynomial=0, scaling_factor=1, generator_start=0, variable_block_length_sgadvanced=, variable_block_length=off, symbols_per_block=255, data_symbols=239, variable_number_of_check_symbols_sgadvanced=, variable_number_of_check_symbols=off, define_supported_r_in_values_sgadvanced=, define_supported_r_in_values=off, number_of_supported_r_in_values=2, supported_r_in_definition_file='no_coe_file_loaded', optimization_sgadvanced=, optimization=Speed, self_recovering_sgadvanced=, self_recovering=off, memory_style=Automatic, clocks_per_symbol=1, number_of_channels=1, number_of_puncture_patterns=0, puncture_definition_file='no_coe_file_loaded', clock_enable_sgadvanced=, clock_enable=off, info_end_sgadvanced=, info_end=off, synchronous_reset_sgadvanced=, synchronous_reset=off, original_delayed_data_sgadvanced=, original_delayed_data=off, erase_sgadvanced=, erase=off, error_statistics_sgadvanced=, error_statistics=off, marker_bits_sgadvanced=, marker_bits=off, number_of_marker_bits=1, ip_name=Reed-Solomon Decoder, ip_version=7.0, dsptool_ready=false, ipcore_usecache=true, ipcore_useipmodelcache=true, wrapper_available=true, port_translation_map={ 'ce' => 'en', 'sr' => 'rst'}, structural_sim=true, ipcore_do_not_force_period=true, has_advanced_control=0, sggui_pos=-1,-1,-1,-1, block_type=rs_decoder_v7_0, block_version=, sg_icon_stat=95,143,2,8,white,green,0,a0c14070,right,,[ ],[ ], sg_mask_display=|, sg_list_contents=, sg_blockgui_xml=}
      mask sg_mask_display=|
      | fprintf('','COMMENT: begin icon graphics');
      | patch([0 95 95 0 0 ],[0 0 143 143 0 ],[0.72 0.84 0.7 ]);
      | plot([0 95 95 0 0 ],[0 0 143 143 0 ]);
      | patch([18.075 36.86 49.86 62.86 75.86 49.86 31.075 18.075 ],[85.43 85.43 98.43 85.43 98.43 98.43 98.43 85.43 ],[1 1 1 ]);
      | patch([31.075 49.86 36.86 18.075 31.075 ],[72.43 72.43 85.43 85.43 72.43 ],[0.916 0.952 0.91 ]);
      | patch([18.075 36.86 49.86 31.075 18.075 ],[59.43 59.43 72.43 72.43 59.43 ],[1 1 1 ]);
      | patch([31.075 75.86 62.86 49.86 36.86 18.075 31.075 ],[46.43 46.43 59.43 46.43 59.43 59.43 46.43 ],[0.916 0.952 0.91 ]);
      | fprintf('','COMMENT: end icon graphics');
      | fprintf('','COMMENT: begin icon text');
      | color('black');port_label('input',1,'data_in');
      | color('black');port_label('input',2,'sync');
      | color('black');port_label('output',1,'data_out');
      | color('black');port_label('output',2,'err_cnt');
      | color('black');port_label('output',3,'err_found');
      | color('black');port_label('output',4,'fail');
      | color('black');port_label('output',5,'blk_strt');
      | color('black');port_label('output',6,'blk_end');
      | color('black');port_label('output',7,'ready');
      | color('black');port_label('output',8,'rffd');
      | fprintf('','COMMENT: end icon text');
      mask prompts: code_specification "Code Specification"; symbol_width "Symbol Width"; field_polynomial "Field Polynomial"; scaling_factor "Scaling Factor (h)"; generator_start "Generator Start"; variable_block_length_sgadvanced ""; variable_block_length "Variable Block Length"; symbols_per_block "Symbols Per Block (n)"; data_symbols "Data Symbols (k)"; variable_number_of_check_symbols_sgadvanced ""; variable_number_of_check_symbols "Variable Number Of Check Symbols (r)"; define_supported_r_in_values_sgadvanced ""; define_supported_r_in_values "Define Supported R_IN Values"; number_of_supported_r_in_values ""; supported_r_in_definition_file ""; optimization_sgadvanced ""; optimization ""; self_recovering_sgadvanced ""; self_recovering "Self Recovering"; memory_style "Memory Style"; clocks_per_symbol "Clocks Per Symbol"; number_of_channels "Number Of Channels"; number_of_puncture_patterns ""; puncture_definition_file ""; clock_enable_sgadvanced ""; clock_enable "Clock Enable"; info_end_sgadvanced ""; info_end "Info End"; synchronous_reset_sgadvanced ""; synchronous_reset "Synchronous Reset"; original_delayed_data_sgadvanced ""; original_delayed_data "Original Delayed Data"; erase_sgadvanced ""; error_statistics_sgadvanced ""; error_statistics "Error Statistics"; marker_bits_sgadvanced ""; marker_bits "Marker Bits"; number_of_marker_bits "Number Of Marker Bits"; ip_name ""; ip_version ""; dsptool_ready ""; ipcore_usecache ""; ipcore_useipmodelcache ""; wrapper_available ""; port_translation_map ""; structural_sim ""; ipcore_do_not_force_period ""; has_advanced_control ""; sggui_pos ""; block_type ""; block_version ""; sg_icon_stat ""; sg_mask_display ""; sg_list_contents ""; sg_blockgui_xml ""
      mask help: Xilinx Reed-Solomon Decoder 7.0
      mask init:
      | try
      |   tmp_gcb = gcb;
      |   tmp_gcbh = gcbh;
      |   if (strcmp('SysGenIndex',get_param(bdroot(tmp_gcbh),'tag')) && ~isempty(regexp(bdroot(tmp_gcb), '^xbs', 'once')))
      |     return;
      |   end;
      |   xlMungeMaskParams;
      |   block_config = 'sysgen:coregenimport_config';
      | 
      |   block_type='rs_decoder_v7_0';
      | 
      |   serialized_declarations = '{''clock_enable''=>''Bool'',''clocks_per_symbol''=>''Int'',''code_specification''=>''String'',''data_symbols''=>''Int'',''define_supported_r_in_values''=>''Bool'',''dsptool_ready''=>''Bool'',''erase''=>''Bool'',''error_statistics''=>''Bool'',''field_polynomial''=>''Int'',''generator_start''=>''Int'',''info_end''=>''Bool'',''ip_name''=>''String'',''ip_version''=>''String'',''ipcore_do_not_force_period''=>''Bool'',''ipcore_usecache''=>''Bool'',''ipcore_useipmodelcache''=>''Bool'',''marker_bits''=>''Bool'',''memory_style''=>''String'',''number_of_channels''=>''Int'',''number_of_marker_bits''=>''Int'',''number_of_puncture_patterns''=>''Int'',''number_of_supported_r_in_values''=>''Int'',''optimization''=>''String'',''original_delayed_data''=>''Bool'',''port_translation_map''=>''String'',''puncture_definition_file''=>''String'',''scaling_factor''=>''Int'',''self_recovering''=>''Bool'',''structural_sim''=>''Bool'',''supported_r_in_definition_file''=>''String'',''symbol_width''=>''String'',''symbols_per_block''=>''Int'',''synchronous_reset''=>''Bool'',''variable_block_length''=>''Bool'',''variable_number_of_check_symbols''=>''Bool'',''wrapper_available''=>''Bool'',''block_type''=>''String''}';
      |   ptable_ = xlblockprep(get_param(tmp_gcb, 'MaskWSVariables'));
      |   try
      |     xlBlockMoveCallback(tmp_gcbh);
      |   catch 
      |      clear global xl_updateicon_recursion_guard;
      |   end;
      | catch
      |   global dbgsysgen;
      |   if(~isempty(dbgsysgen) && dbgsysgen)
      |     e = regexprep(lasterr, '\n', '\nError: ');
      |     disp(['Error: While running MaskInit code on block ' tmp_gcb ': ' e]);
      |     error(e);
      |   end
      | end
      settings: CopyFcn=xlBlockMoveCallback(gcbh);  DeleteFcn=xlDestroyGui(gcbh);  ModelCloseFcn=xlDestroyGui(gcbh);  PreSaveFcn=xlBlockPreSaveCallback(gcbh);  PostSaveFcn=xlBlockPostSaveCallback(gcbh);  DestroyFcn=xlDestroyGui(gcbh);  OpenFcn=xlOpenGui(gcbh, 'rs_decoder_v7_0_gui.xml', @rs_decoder_v7_0_enablement, @rs_decoder_v7_0_action)  CloseFcn=xlDestroyGui(gcbh);  MoveFcn=xlBlockMoveCallback(gcbh);
      mask Help: eval('');xlDoc('-book','sysgen','-topic','Reed_Solomon_Decoder_7_0');
      mask StyleString: popup(Custom|DVB|ATSC|CCSDS|IESS-308(All)|IESS-308(126)|IESS-308(194)|IESS-308(208)|IESS-308(219)|IESS-308(225)|IEEE-802.16),popup(3|4|5|6|7|8|9|10|11|12),edit,edit,edit,edit,checkbox,edit,edit,edit,checkbox,edit,checkbox,edit,edit,edit,popup(Area|Speed),edit,checkbox,popup(Automatic|Block|Distributed),edit,edit,edit,edit,edit,checkbox,edit,checkbox,edit,checkbox,edit,checkbox,edit,checkbox,edit,checkbox,edit,checkbox,edit,edit,edit,edit,edit,edit,edit,edit,edit,edit,edit,edit,edit,edit,edit,edit,edit,edit
      mask Display:
      | fprintf('','COMMENT: begin icon graphics');
      | patch([0 95 95 0 0 ],[0 0 143 143 0 ],[0.72 0.84 0.7 ]);
      | plot([0 95 95 0 0 ],[0 0 143 143 0 ]);
      | patch([18.075 36.86 49.86 62.86 75.86 49.86 31.075 18.075 ],[85.43 85.43 98.43 85.43 98.43 98.43 98.43 85.43 ],[1 1 1 ]);
      | patch([31.075 49.86 36.86 18.075 31.075 ],[72.43 72.43 85.43 85.43 72.43 ],[0.916 0.952 0.91 ]);
      | patch([18.075 36.86 49.86 31.075 18.075 ],[59.43 59.43 72.43 72.43 59.43 ],[1 1 1 ]);
      | patch([31.075 75.86 62.86 49.86 36.86 18.075 31.075 ],[46.43 46.43 59.43 46.43 59.43 59.43 46.43 ],[0.916 0.952 0.91 ]);
      | fprintf('','COMMENT: end icon graphics');
      | fprintf('','COMMENT: begin icon text');
      | color('black');port_label('input',1,'data_in');
      | color('black');port_label('input',2,'sync');
      | color('black');port_label('output',1,'data_out');
      | color('black');port_label('output',2,'err_cnt');
      | color('black');port_label('output',3,'err_found');
      | color('black');port_label('output',4,'fail');
      | color('black');port_label('output',5,'blk_strt');
      | color('black');port_label('output',6,'blk_end');
      | color('black');port_label('output',7,'ready');
      | color('black');port_label('output',8,'rffd');
      | fprintf('','COMMENT: end icon text');
  "Reed-Solomon Decoder 7.1 " : S-Function  LoadFcn=xlBlockLoadCallback(gcbh);  FunctionName=sysgen  Parameters=ptable_  EnableBusSupport=off  mask(Xilinx Reed-Solomon Decoder 7.1  Block){code_specification=Custom, symbol_width=8, field_polynomial=0, scaling_factor=1, generator_start=0, variable_block_length_sgadvanced=, variable_block_length=off, symbols_per_block=255, data_symbols=239, variable_number_of_check_symbols_sgadvanced=, variable_number_of_check_symbols=off, define_supported_r_in_values_sgadvanced=, define_supported_r_in_values=off, number_of_supported_r_in_values=2, supported_r_in_definition_file='no_coe_file_loaded', optimization_sgadvanced=, optimization=Speed, self_recovering_sgadvanced=, self_recovering=off, memory_style=Automatic, clocks_per_symbol=1, number_of_channels=1, number_of_puncture_patterns=0, puncture_definition_file='no_coe_file_loaded', clock_enable_sgadvanced=, clock_enable=off, info_end_sgadvanced=, info_end=off, synchronous_reset_sgadvanced=, synchronous_reset=off, original_delayed_data_sgadvanced=, original_delayed_data=off, erase_sgadvanced=, erase=off, error_statistics_sgadvanced=, error_statistics=off, marker_bits_sgadvanced=, marker_bits=off, number_of_marker_bits=1, ip_name=Reed-Solomon Decoder, ip_version=7.1, dsptool_ready=false, ipcore_usecache=true, ipcore_useipmodelcache=true, wrapper_available=true, port_translation_map={ 'ce' => 'en', 'sr' => 'rst'}, structural_sim=true, ipcore_do_not_force_period=true, has_advanced_control=0, sggui_pos=-1,-1,-1,-1, block_type=rs_decoder_v7_1, block_version=, sg_icon_stat=95,143,2,8,white,green,0,a0c14070,right,,[ ],[ ], sg_mask_display=|, sg_list_contents=, sg_blockgui_xml=}
      mask sg_mask_display=|
      | fprintf('','COMMENT: begin icon graphics');
      | patch([0 95 95 0 0 ],[0 0 143 143 0 ],[0.72 0.84 0.7 ]);
      | plot([0 95 95 0 0 ],[0 0 143 143 0 ]);
      | patch([18.075 36.86 49.86 62.86 75.86 49.86 31.075 18.075 ],[85.43 85.43 98.43 85.43 98.43 98.43 98.43 85.43 ],[1 1 1 ]);
      | patch([31.075 49.86 36.86 18.075 31.075 ],[72.43 72.43 85.43 85.43 72.43 ],[0.916 0.952 0.91 ]);
      | patch([18.075 36.86 49.86 31.075 18.075 ],[59.43 59.43 72.43 72.43 59.43 ],[1 1 1 ]);
      | patch([31.075 75.86 62.86 49.86 36.86 18.075 31.075 ],[46.43 46.43 59.43 46.43 59.43 59.43 46.43 ],[0.916 0.952 0.91 ]);
      | fprintf('','COMMENT: end icon graphics');
      | fprintf('','COMMENT: begin icon text');
      | color('black');port_label('input',1,'data_in');
      | color('black');port_label('input',2,'sync');
      | color('black');port_label('output',1,'data_out');
      | color('black');port_label('output',2,'err_cnt');
      | color('black');port_label('output',3,'err_found');
      | color('black');port_label('output',4,'fail');
      | color('black');port_label('output',5,'blk_strt');
      | color('black');port_label('output',6,'blk_end');
      | color('black');port_label('output',7,'ready');
      | color('black');port_label('output',8,'rffd');
      | fprintf('','COMMENT: end icon text');
      mask prompts: code_specification "Code Specification"; symbol_width "Symbol Width"; field_polynomial "Field Polynomial"; scaling_factor "Scaling Factor (h)"; generator_start "Generator Start"; variable_block_length_sgadvanced ""; variable_block_length "Variable Block Length"; symbols_per_block "Symbols Per Block (n)"; data_symbols "Data Symbols (k)"; variable_number_of_check_symbols_sgadvanced ""; variable_number_of_check_symbols "Variable Number Of Check Symbols (r)"; define_supported_r_in_values_sgadvanced ""; define_supported_r_in_values "Define Supported R_IN Values"; number_of_supported_r_in_values ""; supported_r_in_definition_file ""; optimization_sgadvanced ""; optimization ""; self_recovering_sgadvanced ""; self_recovering "Self Recovering"; memory_style "Memory Style"; clocks_per_symbol "Clocks Per Symbol"; number_of_channels "Number Of Channels"; number_of_puncture_patterns ""; puncture_definition_file ""; clock_enable_sgadvanced ""; clock_enable "Clock Enable"; info_end_sgadvanced ""; info_end "Info End"; synchronous_reset_sgadvanced ""; synchronous_reset "Synchronous Reset"; original_delayed_data_sgadvanced ""; original_delayed_data "Original Delayed Data"; erase_sgadvanced ""; error_statistics_sgadvanced ""; error_statistics "Error Statistics"; marker_bits_sgadvanced ""; marker_bits "Marker Bits"; number_of_marker_bits "Number Of Marker Bits"; ip_name ""; ip_version ""; dsptool_ready ""; ipcore_usecache ""; ipcore_useipmodelcache ""; wrapper_available ""; port_translation_map ""; structural_sim ""; ipcore_do_not_force_period ""; has_advanced_control ""; sggui_pos ""; block_type ""; block_version ""; sg_icon_stat ""; sg_mask_display ""; sg_list_contents ""; sg_blockgui_xml ""
      mask help: Xilinx Reed-Solomon Decoder 7.1
      mask init:
      | try
      |   tmp_gcb = gcb;
      |   tmp_gcbh = gcbh;
      |   if (strcmp('SysGenIndex',get_param(bdroot(tmp_gcbh),'tag')) && ~isempty(regexp(bdroot(tmp_gcb), '^xbs', 'once')))
      |     return;
      |   end;
      |   xlMungeMaskParams;
      |   block_config = 'sysgen:coregenimport_config';
      | 
      |   block_type='rs_decoder_v7_1';
      | 
      |   serialized_declarations = '{''clock_enable''=>''Bool'',''clocks_per_symbol''=>''Int'',''code_specification''=>''String'',''data_symbols''=>''Int'',''define_supported_r_in_values''=>''Bool'',''dsptool_ready''=>''Bool'',''erase''=>''Bool'',''error_statistics''=>''Bool'',''field_polynomial''=>''Int'',''generator_start''=>''Int'',''info_end''=>''Bool'',''ip_name''=>''String'',''ip_version''=>''String'',''ipcore_do_not_force_period''=>''Bool'',''ipcore_usecache''=>''Bool'',''ipcore_useipmodelcache''=>''Bool'',''marker_bits''=>''Bool'',''memory_style''=>''String'',''number_of_channels''=>''Int'',''number_of_marker_bits''=>''Int'',''number_of_puncture_patterns''=>''Int'',''number_of_supported_r_in_values''=>''Int'',''optimization''=>''String'',''original_delayed_data''=>''Bool'',''port_translation_map''=>''String'',''puncture_definition_file''=>''String'',''scaling_factor''=>''Int'',''self_recovering''=>''Bool'',''structural_sim''=>''Bool'',''supported_r_in_definition_file''=>''String'',''symbol_width''=>''String'',''symbols_per_block''=>''Int'',''synchronous_reset''=>''Bool'',''variable_block_length''=>''Bool'',''variable_number_of_check_symbols''=>''Bool'',''wrapper_available''=>''Bool'',''block_type''=>''String''}';
      |   ptable_ = xlblockprep(get_param(tmp_gcb, 'MaskWSVariables'));
      |   try
      |     xlBlockMoveCallback(tmp_gcbh);
      |   catch 
      |      clear global xl_updateicon_recursion_guard;
      |   end;
      | catch
      |   global dbgsysgen;
      |   if(~isempty(dbgsysgen) && dbgsysgen)
      |     e = regexprep(lasterr, '\n', '\nError: ');
      |     disp(['Error: While running MaskInit code on block ' tmp_gcb ': ' e]);
      |     error(e);
      |   end
      | end
      settings: CopyFcn=xlBlockMoveCallback(gcbh);  DeleteFcn=xlDestroyGui(gcbh);  ModelCloseFcn=xlDestroyGui(gcbh);  PreSaveFcn=xlBlockPreSaveCallback(gcbh);  PostSaveFcn=xlBlockPostSaveCallback(gcbh);  DestroyFcn=xlDestroyGui(gcbh);  OpenFcn=xlOpenGui(gcbh, 'rs_decoder_v7_1_gui.xml', @rs_decoder_v7_1_enablement, @rs_decoder_v7_1_action)  CloseFcn=xlDestroyGui(gcbh);  MoveFcn=xlBlockMoveCallback(gcbh);
      mask Help: eval('');xlDoc('-book','sysgen','-topic','Reed_Solomon_Decoder_7_1');
      mask StyleString: popup(Custom|DVB|ATSC|CCSDS|IESS-308(All)|IESS-308(126)|IESS-308(194)|IESS-308(208)|IESS-308(219)|IESS-308(225)|IEEE-802.16),popup(3|4|5|6|7|8|9|10|11|12),edit,edit,edit,edit,checkbox,edit,edit,edit,checkbox,edit,checkbox,edit,edit,edit,popup(Area|Speed),edit,checkbox,popup(Automatic|Block|Distributed),edit,edit,edit,edit,edit,checkbox,edit,checkbox,edit,checkbox,edit,checkbox,edit,checkbox,edit,checkbox,edit,checkbox,edit,edit,edit,edit,edit,edit,edit,edit,edit,edit,edit,edit,edit,edit,edit,edit,edit,edit
      mask Display:
      | fprintf('','COMMENT: begin icon graphics');
      | patch([0 95 95 0 0 ],[0 0 143 143 0 ],[0.72 0.84 0.7 ]);
      | plot([0 95 95 0 0 ],[0 0 143 143 0 ]);
      | patch([18.075 36.86 49.86 62.86 75.86 49.86 31.075 18.075 ],[85.43 85.43 98.43 85.43 98.43 98.43 98.43 85.43 ],[1 1 1 ]);
      | patch([31.075 49.86 36.86 18.075 31.075 ],[72.43 72.43 85.43 85.43 72.43 ],[0.916 0.952 0.91 ]);
      | patch([18.075 36.86 49.86 31.075 18.075 ],[59.43 59.43 72.43 72.43 59.43 ],[1 1 1 ]);
      | patch([31.075 75.86 62.86 49.86 36.86 18.075 31.075 ],[46.43 46.43 59.43 46.43 59.43 59.43 46.43 ],[0.916 0.952 0.91 ]);
      | fprintf('','COMMENT: end icon graphics');
      | fprintf('','COMMENT: begin icon text');
      | color('black');port_label('input',1,'data_in');
      | color('black');port_label('input',2,'sync');
      | color('black');port_label('output',1,'data_out');
      | color('black');port_label('output',2,'err_cnt');
      | color('black');port_label('output',3,'err_found');
      | color('black');port_label('output',4,'fail');
      | color('black');port_label('output',5,'blk_strt');
      | color('black');port_label('output',6,'blk_end');
      | color('black');port_label('output',7,'ready');
      | color('black');port_label('output',8,'rffd');
      | fprintf('','COMMENT: end icon text');
  "Reed-Solomon Decoder 8.0 " : S-Function  LoadFcn=xlBlockLoadCallback(gcbh);  FunctionName=sysgen  Parameters=ptable_  EnableBusSupport=off  mask(Xilinx Reed-Solomon Decoder 8.0  Block){code_specification=Custom, symbol_width=8, field_polynomial=0, scaling_factor=1, generator_start=0, variable_block_length_sgadvanced=, variable_block_length=off, symbols_per_block=255, data_symbols=239, variable_number_of_check_symbols_sgadvanced=, variable_number_of_check_symbols=off, define_supported_r_in_values_sgadvanced=, define_supported_r_in_values=off, number_of_supported_r_in_values=2, supported_r_in_definition_file='no_coe_file_loaded', self_recovering_sgadvanced=, self_recovering=off, memory_style=Automatic, number_of_channels=1, output_check_symbols=on, number_of_puncture_patterns=0, puncture_definition_file='no_coe_file_loaded', aclken_sgadvanced=, aclken=off, info_sgadvanced=, info=off, aresetn_sgadvanced=, aresetn=off, original_delayed_data_sgadvanced=, original_delayed_data=off, erase_sgadvanced=, erase=off, error_statistics_sgadvanced=, error_statistics=off, marker_bits_sgadvanced=, marker_bits=off, number_of_marker_bits=1, trim_axipin_name=on, ip_name=Reed-Solomon Decoder, ip_version=8.0, dsptool_ready=false, ipcore_usecache=true, ipcore_useipmodelcache=true, wrapper_available=true, port_translation_map={ 'aclken' => 'en', 'aresetn' => 'rst'}, structural_sim=true, ipcore_do_not_force_period=true, has_advanced_control=0, sggui_pos=-1,-1,-1,-1, block_type=rs_decoder_v8_0, block_version=, sg_icon_stat=95,142,5,11,white,green,0,b04947a5,right,,[2 2 2 3 4 ],[2 3 3 3 4 4 4 4 1 1 1 ], sg_mask_display=|, sg_list_contents=, sg_blockgui_xml=}
      mask sg_mask_display=|
      | fprintf('','COMMENT: begin icon graphics');
      | patch([0 0 2 2 ],[142 60 60 142 ],[5.650000e-001 6.550000e-001 5.500000e-001 ]);
      | patch([0 0 2 2 ],[52 30 30 52 ],[4.100000e-001 4.700000e-001 4.000000e-001 ]);
      | patch([0 0 2 2 ],[22 0 0 22 ],[2.550000e-001 2.850000e-001 2.500000e-001 ]);
      | patch([93 93 95 95 ],[125 117 117 125 ],[5.650000e-001 6.550000e-001 5.500000e-001 ]);
      | patch([93 93 95 95 ],[115 87 87 115 ],[4.100000e-001 4.700000e-001 4.000000e-001 ]);
      | patch([93 93 95 95 ],[85 47 47 85 ],[2.550000e-001 2.850000e-001 2.500000e-001 ]);
      | patch([93 93 95 95 ],[45 17 17 45 ],[7.200000e-001 8.400000e-001 7.000000e-001 ]);
      | patch([2 92 92 2 2 ],[0 0 142 142 0 ],[7.200000e-001 8.400000e-001 7.000000e-001 ]);
      | plot([2 92 92 2 2 ],[0 0 142 142 0 ]);
      |
      |
      | patch([18.075 36.86 49.86 62.86 75.86 49.86 31.075 18.075 ],[85.43 85.43 98.43 85.43 98.43 98.43 98.43 85.43 ],[1 1 1 ]);
      | patch([31.075 49.86 36.86 18.075 31.075 ],[72.43 72.43 85.43 85.43 72.43 ],[0.916 0.952 0.91 ]);
      | patch([18.075 36.86 49.86 31.075 18.075 ],[59.43 59.43 72.43 72.43 59.43 ],[1 1 1 ]);
      | patch([31.075 75.86 62.86 49.86 36.86 18.075 31.075 ],[46.43 46.43 59.43 46.43 59.43 59.43 46.43 ],[0.916 0.952 0.91 ]);
      | fprintf('','COMMENT: end icon graphics');
      | fprintf('','COMMENT: begin icon text');
      | color('black');port_label('input',1,'  input_tvalid  ');
      | color('black');port_label('input',2,'  input_tdata_data_in  ');
      | color('black');port_label('input',3,'  input_tlast  ');
      | color('black');port_label('input',4,'  output_tready  ');
      | color('black');port_label('input',5,'  stat_tready  ');
      | color('black');port_label('output',1,'  input_tready  ');
      | color('black');port_label('output',2,'  output_tvalid  ');
      | color('black');port_label('output',3,'  output_tdata_data_out  ');
      | color('black');port_label('output',4,'  output_tlast  ');
      | color('black');port_label('output',5,'  stat_tvalid  ');
      | color('black');port_label('output',6,'  stat_tdata_err_cnt  ');
      | color('black');port_label('output',7,'  stat_tdata_err_found  ');
      | color('black');port_label('output',8,'  stat_tdata_fail  ');
      | color('black');port_label('output',9,'  event_s_input_tlast_missing  ');
      | color('black');port_label('output',10,'  event_s_input_tlast_unexpected  ');
      | color('black');port_label('output',11,'  event_s_ctrl_tdata_invalid  ');
      | fprintf('','COMMENT: end icon text');
      mask prompts: code_specification "Code Specification"; symbol_width "Symbol Width"; field_polynomial "Field Polynomial"; scaling_factor "Scaling Factor (h)"; generator_start "Generator Start"; variable_block_length_sgadvanced ""; variable_block_length "Variable Block Length"; symbols_per_block "Symbols Per Block (n)"; data_symbols "Data Symbols (k)"; variable_number_of_check_symbols_sgadvanced ""; variable_number_of_check_symbols "Variable Number Of Check Symbols (r)"; define_supported_r_in_values_sgadvanced ""; define_supported_r_in_values "Define Supported R_IN Values"; number_of_supported_r_in_values ""; supported_r_in_definition_file ""; self_recovering_sgadvanced ""; self_recovering "Self Recovering"; memory_style "Memory Style"; number_of_channels "Number Of Channels"; output_check_symbols "Output check symbols (Output all N symbols in block, including check symbols, or only K information symbols)"; number_of_puncture_patterns ""; puncture_definition_file ""; aclken_sgadvanced ""; aclken "Clock Enable"; info_sgadvanced ""; aresetn_sgadvanced ""; aresetn "Synchronous Reset"; original_delayed_data_sgadvanced ""; original_delayed_data "Original Delayed Data"; erase_sgadvanced ""; error_statistics_sgadvanced ""; error_statistics "Error Statistics"; marker_bits_sgadvanced ""; marker_bits "Marker Bits"; number_of_marker_bits "Number Of Marker Bits"; trim_axipin_name "Display shortened port names"; ip_name ""; ip_version ""; dsptool_ready ""; ipcore_usecache ""; ipcore_useipmodelcache ""; wrapper_available ""; port_translation_map ""; structural_sim ""; ipcore_do_not_force_period ""; has_advanced_control ""; sggui_pos ""; block_type ""; block_version ""; sg_icon_stat ""; sg_mask_display ""; sg_list_contents ""; sg_blockgui_xml ""
      mask help: Xilinx Reed-Solomon Decoder 8.0
